simulink model "Masse_MultirotorSimHinf"  (R2018b)
settings: Solver=VariableStepAuto  StartTime=0.0  StopTime=Simulation.T_END  MaxStep=Simulation.TS_MAX  RelTol=1e-3  EnableMultiTasking=on
PreLoadFcn:
  | % InitializeParameters;
undefined symbols (not defined in the file): Aero, armed, ctrl_state, INIT_PARAM_VECTOR, Initial, K_i, K_p, Motor, mpc_att_sp, mpc_ctrl_state, mpc_manual, mpc_pos_sp_triplet, mpc_vehicle_land_detected, mpc_vehicle_status, Simulation, SOF1, SOF2, Uav, Upsilon, v_att_sp, v_control_mode
libraries: simulink_extras x9, simulink x6, dspstat3 x1, Px4Library x1
(part 4 of 11)

== matlab function Masse_MultirotorSimHinf/Sensor Model/local_position_estimator/local_position_estimator ==
  data: time input; selfVecIn input; selfVecOut output; LPE_SAMPLING_PERIOD parameter
function selfVecOut  = lpeMain( time, selfVecIn, LPE_SAMPLING_PERIOD )
%#codegen
	self = DecodeSelf( selfVecIn );
	self = LocalPositionEstimator( self, time*1e6, LPE_SAMPLING_PERIOD );
	selfVecOut = EncodeSelf( self );
end

function self = DecodeSelf( selfVecIn )
	% Variable assignment
	                                  self.A        = zeros(10,10);
	                                  self.A( 1, 1) = selfVecIn(  1);
	                                  self.A( 1, 2) = selfVecIn(  2);
	                                  self.A( 1, 3) = selfVecIn(  3);
	                                  self.A( 1, 4) = selfVecIn(  4);
	                                  self.A( 1, 5) = selfVecIn(  5);
	                                  self.A( 1, 6) = selfVecIn(  6);
	                                  self.A( 1, 7) = selfVecIn(  7);
	                                  self.A( 1, 8) = selfVecIn(  8);
	                                  self.A( 1, 9) = selfVecIn(  9);
	                                  self.A( 1,10) = selfVecIn( 10);
	                                  self.A( 2, 1) = selfVecIn( 11);
	                                  self.A( 2, 2) = selfVecIn( 12);
	                                  self.A( 2, 3) = selfVecIn( 13);
	                                  self.A( 2, 4) = selfVecIn( 14);
	                                  self.A( 2, 5) = selfVecIn( 15);
	                                  self.A( 2, 6) = selfVecIn( 16);
	                                  self.A( 2, 7) = selfVecIn( 17);
	                                  self.A( 2, 8) = selfVecIn( 18);
	                                  self.A( 2, 9) = selfVecIn( 19);
	                                  self.A( 2,10) = selfVecIn( 20);
	                                  self.A( 3, 1) = selfVecIn( 21);
	                                  self.A( 3, 2) = selfVecIn( 22);
	                                  self.A( 3, 3) = selfVecIn( 23);
	                                  self.A( 3, 4) = selfVecIn( 24);
	                                  self.A( 3, 5) = selfVecIn( 25);
	                                  self.A( 3, 6) = selfVecIn( 26);
	                                  self.A( 3, 7) = selfVecIn( 27);
	                                  self.A( 3, 8) = selfVecIn( 28);
	                                  self.A( 3, 9) = selfVecIn( 29);
	                                  self.A( 3,10) = selfVecIn( 30);
	                                  self.A( 4, 1) = selfVecIn( 31);
	                                  self.A( 4, 2) = selfVecIn( 32);
	                                  self.A( 4, 3) = selfVecIn( 33);
	                                  self.A( 4, 4) = selfVecIn( 34);
	                                  self.A( 4, 5) = selfVecIn( 35);
	                                  self.A( 4, 6) = selfVecIn( 36);
	                                  self.A( 4, 7) = selfVecIn( 37);
	                                  self.A( 4, 8) = selfVecIn( 38);
	                                  self.A( 4, 9) = selfVecIn( 39);
	                                  self.A( 4,10) = selfVecIn( 40);
	                                  self.A( 5, 1) = selfVecIn( 41);
	                                  self.A( 5, 2) = selfVecIn( 42);
	                                  self.A( 5, 3) = selfVecIn( 43);
	                                  self.A( 5, 4) = selfVecIn( 44);
	                                  self.A( 5, 5) = selfVecIn( 45);
	                                  self.A( 5, 6) = selfVecIn( 46);
	                                  self.A( 5, 7) = selfVecIn( 47);
	                                  self.A( 5, 8) = selfVecIn( 48);
	                                  self.A( 5, 9) = selfVecIn( 49);
	                                  self.A( 5,10) = selfVecIn( 50);
	                                  self.A( 6, 1) = selfVecIn( 51);
	                                  self.A( 6, 2) = selfVecIn( 52);
	                                  self.A( 6, 3) = selfVecIn( 53);
	                                  self.A( 6, 4) = selfVecIn( 54);
	                                  self.A( 6, 5) = selfVecIn( 55);
	                                  self.A( 6, 6) = selfVecIn( 56);
	                                  self.A( 6, 7) = selfVecIn( 57);
	                                  self.A( 6, 8) = selfVecIn( 58);
	                                  self.A( 6, 9) = selfVecIn( 59);
	                                  self.A( 6,10) = selfVecIn( 60);
	                                  self.A( 7, 1) = selfVecIn( 61);
	                                  self.A( 7, 2) = selfVecIn( 62);
	                                  self.A( 7, 3) = selfVecIn( 63);
	                                  self.A( 7, 4) = selfVecIn( 64);
	                                  self.A( 7, 5) = selfVecIn( 65);
	                                  self.A( 7, 6) = selfVecIn( 66);
	                                  self.A( 7, 7) = selfVecIn( 67);
	                                  self.A( 7, 8) = selfVecIn( 68);
	                                  self.A( 7, 9) = selfVecIn( 69);
	                                  self.A( 7,10) = selfVecIn( 70);
	                                  self.A( 8, 1) = selfVecIn( 71);
	                                  self.A( 8, 2) = selfVecIn( 72);
	                                  self.A( 8, 3) = selfVecIn( 73);
	                                  self.A( 8, 4) = selfVecIn( 74);
	                                  self.A( 8, 5) = selfVecIn( 75);
	                                  self.A( 8, 6) = selfVecIn( 76);
	                                  self.A( 8, 7) = selfVecIn( 77);
	                                  self.A( 8, 8) = selfVecIn( 78);
	                                  self.A( 8, 9) = selfVecIn( 79);
	                                  self.A( 8,10) = selfVecIn( 80);
	                                  self.A( 9, 1) = selfVecIn( 81);
	                                  self.A( 9, 2) = selfVecIn( 82);
	                                  self.A( 9, 3) = selfVecIn( 83);
	                                  self.A( 9, 4) = selfVecIn( 84);
	                                  self.A( 9, 5) = selfVecIn( 85);
	                                  self.A( 9, 6) = selfVecIn( 86);
	                                  self.A( 9, 7) = selfVecIn( 87);
	                                  self.A( 9, 8) = selfVecIn( 88);
	                                  self.A( 9, 9) = selfVecIn( 89);
	                                  self.A( 9,10) = selfVecIn( 90);
	                                  self.A(10, 1) = selfVecIn( 91);
	                                  self.A(10, 2) = selfVecIn( 92);
	                                  self.A(10, 3) = selfVecIn( 93);
	                                  self.A(10, 4) = selfVecIn( 94);
	                                  self.A(10, 5) = selfVecIn( 95);
	                                  self.A(10, 6) = selfVecIn( 96);
	                                  self.A(10, 7) = selfVecIn( 97);
	                                  self.A(10, 8) = selfVecIn( 98);
	                                  self.A(10, 9) = selfVecIn( 99);
	                                  self.A(10,10) = selfVecIn(100);
	                                  self.B        = zeros(10, 3);
	                                  self.B( 1, 1) = selfVecIn(101);
	                                  self.B( 1, 2) = selfVecIn(102);
	                                  self.B( 1, 3) = selfVecIn(103);
	                                  self.B( 2, 1) = selfVecIn(104);
	                                  self.B( 2, 2) = selfVecIn(105);
	                                  self.B( 2, 3) = selfVecIn(106);
	                                  self.B( 3, 1) = selfVecIn(107);
	                                  self.B( 3, 2) = selfVecIn(108);
	                                  self.B( 3, 3) = selfVecIn(109);
	                                  self.B( 4, 1) = selfVecIn(110);
	                                  self.B( 4, 2) = selfVecIn(111);
	                                  self.B( 4, 3) = selfVecIn(112);
	                                  self.B( 5, 1) = selfVecIn(113);
	                                  self.B( 5, 2) = selfVecIn(114);
	                                  self.B( 5, 3) = selfVecIn(115);
	                                  self.B( 6, 1) = selfVecIn(116);
	                                  self.B( 6, 2) = selfVecIn(117);
	                                  self.B( 6, 3) = selfVecIn(118);
	                                  self.B( 7, 1) = selfVecIn(119);
	                                  self.B( 7, 2) = selfVecIn(120);
	                                  self.B( 7, 3) = selfVecIn(121);
	                                  self.B( 8, 1) = selfVecIn(122);
	                                  self.B( 8, 2) = selfVecIn(123);
	                                  self.B( 8, 3) = selfVecIn(124);
	                                  self.B( 9, 1) = selfVecIn(125);
	                                  self.B( 9, 2) = selfVecIn(126);
	                                  self.B( 9, 3) = selfVecIn(127);
	                                  self.B(10, 1) = selfVecIn(128);
	                                  self.B(10, 2) = selfVecIn(129);
	                                  self.B(10, 3) = selfVecIn(130);
	                         self.BETA_TABLE        = zeros( 7, 1);
	                         self.BETA_TABLE( 1, 1) = selfVecIn(131);
	                         self.BETA_TABLE( 2, 1) = selfVecIn(132);
	                         self.BETA_TABLE( 3, 1) = selfVecIn(133);
	                         self.BETA_TABLE( 4, 1) = selfVecIn(134);
	                         self.BETA_TABLE( 5, 1) = selfVecIn(135);
	                         self.BETA_TABLE( 6, 1) = selfVecIn(136);
	                         self.BETA_TABLE( 7, 1) = selfVecIn(137);
	                           self.BIAS_MAX        = selfVecIn(138);
	                self.EST_STDDEV_TZ_VALID        = selfVecIn(139);
	                self.EST_STDDEV_XY_VALID        = selfVecIn(140);
	                 self.EST_STDDEV_Z_VALID        = selfVecIn(141);
	                             self.EST_TZ        = uint8(selfVecIn(142));
	                             self.EST_XY        = uint8(selfVecIn(143));
	                              self.EST_Z        = uint8(selfVecIn(144));
	                          self.FUSE_BARO        = uint8(selfVecIn(145));
	                          self.FUSE_FLOW        = uint8(selfVecIn(146));
	                self.FUSE_FLOW_GYRO_COMP        = uint8(selfVecIn(147));
	                           self.FUSE_GPS        = uint8(selfVecIn(148));
	                          self.FUSE_LAND        = uint8(selfVecIn(149));
	                     self.FUSE_PUB_AGL_Z        = uint8(selfVecIn(150));
	                       self.FUSE_VIS_POS        = uint8(selfVecIn(151));
	                       self.FUSE_VIS_YAW        = uint8(selfVecIn(152));
	                          self.HIST_STEP        = selfVecIn(153);
	                          self.LAND_RATE        = selfVecIn(154);
	                                  self.P        = zeros(10,10);
	                                  self.P( 1, 1) = selfVecIn(155);
	                                  self.P( 1, 2) = selfVecIn(156);
	                                  self.P( 1, 3) = selfVecIn(157);
	                                  self.P( 1, 4) = selfVecIn(158);
	                                  self.P( 1, 5) = selfVecIn(159);
	                                  self.P( 1, 6) = selfVecIn(160);
	                                  self.P( 1, 7) = selfVecIn(161);
	                                  self.P( 1, 8) = selfVecIn(162);
	                                  self.P( 1, 9) = selfVecIn(163);
	                                  self.P( 1,10) = selfVecIn(164);
	                                  self.P( 2, 1) = selfVecIn(165);
	                                  self.P( 2, 2) = selfVecIn(166);
	                                  self.P( 2, 3) = selfVecIn(167);
	                                  self.P( 2, 4) = selfVecIn(168);
	                                  self.P( 2, 5) = selfVecIn(169);
	                                  self.P( 2, 6) = selfVecIn(170);
	                                  self.P( 2, 7) = selfVecIn(171);
	                                  self.P( 2, 8) = selfVecIn(172);
	                                  self.P( 2, 9) = selfVecIn(173);
	                                  self.P( 2,10) = selfVecIn(174);
	                                  self.P( 3, 1) = selfVecIn(175);
	                                  self.P( 3, 2) = selfVecIn(176);
	                                  self.P( 3, 3) = selfVecIn(177);
	                                  self.P( 3, 4) = selfVecIn(178);
	                                  self.P( 3, 5) = selfVecIn(179);
	                                  self.P( 3, 6) = selfVecIn(180);
	                                  self.P( 3, 7) = selfVecIn(181);
	                                  self.P( 3, 8) = selfVecIn(182);
	                                  self.P( 3, 9) = selfVecIn(183);
	                                  self.P( 3,10) = selfVecIn(184);
	                                  self.P( 4, 1) = selfVecIn(185);
	                                  self.P( 4, 2) = selfVecIn(186);
	                                  self.P( 4, 3) = selfVecIn(187);
	                                  self.P( 4, 4) = selfVecIn(188);
	                                  self.P( 4, 5) = selfVecIn(189);
	                                  self.P( 4, 6) = selfVecIn(190);
	                                  self.P( 4, 7) = selfVecIn(191);
	                                  self.P( 4, 8) = selfVecIn(192);
	                                  self.P( 4, 9) = selfVecIn(193);
	                                  self.P( 4,10) = selfVecIn(194);
	                                  self.P( 5, 1) = selfVecIn(195);
	                                  self.P( 5, 2) = selfVecIn(196);
	                                  self.P( 5, 3) = selfVecIn(197);
	                                  self.P( 5, 4) = selfVecIn(198);
	                                  self.P( 5, 5) = selfVecIn(199);
	                                  self.P( 5, 6) = selfVecIn(200);
	                                  self.P( 5, 7) = selfVecIn(201);
	                                  self.P( 5, 8) = selfVecIn(202);
	                                  self.P( 5, 9) = selfVecIn(203);
	                                  self.P( 5,10) = selfVecIn(204);
	                                  self.P( 6, 1) = selfVecIn(205);
	                                  self.P( 6, 2) = selfVecIn(206);
	                                  self.P( 6, 3) = selfVecIn(207);
	                                  self.P( 6, 4) = selfVecIn(208);
	                                  self.P( 6, 5) = selfVecIn(209);
	                                  self.P( 6, 6) = selfVecIn(210);
	                                  self.P( 6, 7) = selfVecIn(211);
	                                  self.P( 6, 8) = selfVecIn(212);
	                                  self.P( 6, 9) = selfVecIn(213);
	                                  self.P( 6,10) = selfVecIn(214);
	                                  self.P( 7, 1) = selfVecIn(215);
	                                  self.P( 7, 2) = selfVecIn(216);
	                                  self.P( 7, 3) = selfVecIn(217);
	                                  self.P( 7, 4) = selfVecIn(218);
	                                  self.P( 7, 5) = selfVecIn(219);
	                                  self.P( 7, 6) = selfVecIn(220);
	                                  self.P( 7, 7) = selfVecIn(221);
	                                  self.P( 7, 8) = selfVecIn(222);
	                                  self.P( 7, 9) = selfVecIn(223);
	                                  self.P( 7,10) = selfVecIn(224);
	                                  self.P( 8, 1) = selfVecIn(225);
	                                  self.P( 8, 2) = selfVecIn(226);
	                                  self.P( 8, 3) = selfVecIn(227);
	                                  self.P( 8, 4) = selfVecIn(228);
	                                  self.P( 8, 5) = selfVecIn(229);
	                                  self.P( 8, 6) = selfVecIn(230);
	                                  self.P( 8, 7) = selfVecIn(231);
	                                  self.P( 8, 8) = selfVecIn(232);
	                                  self.P( 8, 9) = selfVecIn(233);
	                                  self.P( 8,10) = selfVecIn(234);
	                                  self.P( 9, 1) = selfVecIn(235);
	                                  self.P( 9, 2) = selfVecIn(236);
	                                  self.P( 9, 3) = selfVecIn(237);
	                                  self.P( 9, 4) = selfVecIn(238);
	                                  self.P( 9, 5) = selfVecIn(239);
	                                  self.P( 9, 6) = selfVecIn(240);
	                                  self.P( 9, 7) = selfVecIn(241);
	                                  self.P( 9, 8) = selfVecIn(242);
	                                  self.P( 9, 9) = selfVecIn(243);
	                                  self.P( 9,10) = selfVecIn(244);
	                                  self.P(10, 1) = selfVecIn(245);
	                                  self.P(10, 2) = selfVecIn(246);
	                                  self.P(10, 3) = selfVecIn(247);
	                                  self.P(10, 4) = selfVecIn(248);
	                                  self.P(10, 5) = selfVecIn(249);
	                                  self.P(10, 6) = selfVecIn(250);
	                                  self.P(10, 7) = selfVecIn(251);
	                                  self.P(10, 8) = selfVecIn(252);
	                                  self.P(10, 9) = selfVecIn(253);
	                                  self.P(10,10) = selfVecIn(254);
	                              self.P_MAX        = selfVecIn(255);
	                                  self.Q        = zeros(10,10);
	                                  self.Q( 1, 1) = selfVecIn(256);
	                                  self.Q( 1, 2) = selfVecIn(257);
	                                  self.Q( 1, 3) = selfVecIn(258);
	                                  self.Q( 1, 4) = selfVecIn(259);
	                                  self.Q( 1, 5) = selfVecIn(260);
	                                  self.Q( 1, 6) = selfVecIn(261);
	                                  self.Q( 1, 7) = selfVecIn(262);
	                                  self.Q( 1, 8) = selfVecIn(263);
	                                  self.Q( 1, 9) = selfVecIn(264);
	                                  self.Q( 1,10) = selfVecIn(265);
	                                  self.Q( 2, 1) = selfVecIn(266);
	                                  self.Q( 2, 2) = selfVecIn(267);
	                                  self.Q( 2, 3) = selfVecIn(268);
	                                  self.Q( 2, 4) = selfVecIn(269);
	                                  self.Q( 2, 5) = selfVecIn(270);
	                                  self.Q( 2, 6) = selfVecIn(271);
	                                  self.Q( 2, 7) = selfVecIn(272);
	                                  self.Q( 2, 8) = selfVecIn(273);
	                                  self.Q( 2, 9) = selfVecIn(274);
	                                  self.Q( 2,10) = selfVecIn(275);
	                                  self.Q( 3, 1) = selfVecIn(276);
	                                  self.Q( 3, 2) = selfVecIn(277);
	                                  self.Q( 3, 3) = selfVecIn(278);
	                                  self.Q( 3, 4) = selfVecIn(279);
	                                  self.Q( 3, 5) = selfVecIn(280);
	                                  self.Q( 3, 6) = selfVecIn(281);
	                                  self.Q( 3, 7) = selfVecIn(282);
	                                  self.Q( 3, 8) = selfVecIn(283);
	                                  self.Q( 3, 9) = selfVecIn(284);
	                                  self.Q( 3,10) = selfVecIn(285);
	                                  self.Q( 4, 1) = selfVecIn(286);
	                                  self.Q( 4, 2) = selfVecIn(287);
	                                  self.Q( 4, 3) = selfVecIn(288);
	                                  self.Q( 4, 4) = selfVecIn(289);
	                                  self.Q( 4, 5) = selfVecIn(290);
	                                  self.Q( 4, 6) = selfVecIn(291);
	                                  self.Q( 4, 7) = selfVecIn(292);
	                                  self.Q( 4, 8) = selfVecIn(293);
	                                  self.Q( 4, 9) = selfVecIn(294);
	                                  self.Q( 4,10) = selfVecIn(295);
	                                  self.Q( 5, 1) = selfVecIn(296);
	                                  self.Q( 5, 2) = selfVecIn(297);
	                                  self.Q( 5, 3) = selfVecIn(298);
	                                  self.Q( 5, 4) = selfVecIn(299);
	                                  self.Q( 5, 5) = selfVecIn(300);
	                                  self.Q( 5, 6) = selfVecIn(301);
	                                  self.Q( 5, 7) = selfVecIn(302);
	                                  self.Q( 5, 8) = selfVecIn(303);
	                                  self.Q( 5, 9) = selfVecIn(304);
	                                  self.Q( 5,10) = selfVecIn(305);
	                                  self.Q( 6, 1) = selfVecIn(306);
	                                  self.Q( 6, 2) = selfVecIn(307);
	                                  self.Q( 6, 3) = selfVecIn(308);
	                                  self.Q( 6, 4) = selfVecIn(309);
	                                  self.Q( 6, 5) = selfVecIn(310);
	                                  self.Q( 6, 6) = selfVecIn(311);
	                                  self.Q( 6, 7) = selfVecIn(312);
	                                  self.Q( 6, 8) = selfVecIn(313);
	                                  self.Q( 6, 9) = selfVecIn(314);
	                                  self.Q( 6,10) = selfVecIn(315);
	                                  self.Q( 7, 1) = selfVecIn(316);
	                                  self.Q( 7, 2) = selfVecIn(317);
	                                  self.Q( 7, 3) = selfVecIn(318);
	                                  self.Q( 7, 4) = selfVecIn(319);
	                                  self.Q( 7, 5) = selfVecIn(320);
	                                  self.Q( 7, 6) = selfVecIn(321);
	                                  self.Q( 7, 7) = selfVecIn(322);
	                                  self.Q( 7, 8) = selfVecIn(323);
	                                  self.Q( 7, 9) = selfVecIn(324);
	                                  self.Q( 7,10) = selfVecIn(325);
	                                  self.Q( 8, 1) = selfVecIn(326);
	                                  self.Q( 8, 2) = selfVecIn(327);
	                                  self.Q( 8, 3) = selfVecIn(328);
	                                  self.Q( 8, 4) = selfVecIn(329);
	                                  self.Q( 8, 5) = selfVecIn(330);
	                                  self.Q( 8, 6) = selfVecIn(331);
	                                  self.Q( 8, 7) = selfVecIn(332);
	                                  self.Q( 8, 8) = selfVecIn(333);
	                                  self.Q( 8, 9) = selfVecIn(334);
	                                  self.Q( 8,10) = selfVecIn(335);
	                                  self.Q( 9, 1) = selfVecIn(336);
	                                  self.Q( 9, 2) = selfVecIn(337);
	                                  self.Q( 9, 3) = selfVecIn(338);
	                                  self.Q( 9, 4) = selfVecIn(339);
	                                  self.Q( 9, 5) = selfVecIn(340);
	                                  self.Q( 9, 6) = selfVecIn(341);
	                                  self.Q( 9, 7) = selfVecIn(342);
	                                  self.Q( 9, 8) = selfVecIn(343);
	                                  self.Q( 9, 9) = selfVecIn(344);
	                                  self.Q( 9,10) = selfVecIn(345);
	                                  self.Q(10, 1) = selfVecIn(346);
	                                  self.Q(10, 2) = selfVecIn(347);
	                                  self.Q(10, 3) = selfVecIn(348);
	                                  self.Q(10, 4) = selfVecIn(349);
	                                  self.Q(10, 5) = selfVecIn(350);
	                                  self.Q(10, 6) = selfVecIn(351);
	                                  self.Q(10, 7) = selfVecIn(352);
	                                  self.Q(10, 8) = selfVecIn(353);
	                                  self.Q(10, 9) = selfVecIn(354);
	                                  self.Q(10,10) = selfVecIn(355);
	                                  self.R        = zeros( 3, 3);
	                                  self.R( 1, 1) = selfVecIn(356);
	                                  self.R( 1, 2) = selfVecIn(357);
	                                  self.R( 1, 3) = selfVecIn(358);
	                                  self.R( 2, 1) = selfVecIn(359);
	                                  self.R( 2, 2) = selfVecIn(360);
	                                  self.R( 2, 3) = selfVecIn(361);
	                                  self.R( 3, 1) = selfVecIn(362);
	                                  self.R( 3, 2) = selfVecIn(363);
	                                  self.R( 3, 3) = selfVecIn(364);
	                              self.R_att        = zeros( 3, 3);
	                              self.R_att( 1, 1) = selfVecIn(365);
	                              self.R_att( 1, 2) = selfVecIn(366);
	                              self.R_att( 1, 3) = selfVecIn(367);
	                              self.R_att( 2, 1) = selfVecIn(368);
	                              self.R_att( 2, 2) = selfVecIn(369);
	                              self.R_att( 2, 3) = selfVecIn(370);
	                              self.R_att( 3, 1) = selfVecIn(371);
	                              self.R_att( 3, 2) = selfVecIn(372);
	                              self.R_att( 3, 3) = selfVecIn(373);
	                        self.SENSOR_BARO        = uint8(selfVecIn(374));
	                        self.SENSOR_FLOW        = uint8(selfVecIn(375));
	                         self.SENSOR_GPS        = uint8(selfVecIn(376));
	                        self.SENSOR_LAND        = uint8(selfVecIn(377));
	                       self.SENSOR_LIDAR        = uint8(selfVecIn(378));
	                       self.SENSOR_MOCAP        = uint8(selfVecIn(379));
	                       self.SENSOR_SONAR        = uint8(selfVecIn(380));
	                      self.SENSOR_VISION        = uint8(selfVecIn(381));
	                    self.accel_xy_stddev        = selfVecIn(382);
	                    self.accel_xy_stddev        = selfVecIn(383);
	                     self.accel_z_stddev        = selfVecIn(384);
	                     self.accel_z_stddev        = selfVecIn(385);
	                      self.aglLowPass.dt        = selfVecIn(386);
	                    self.aglLowPass.fcut        = selfVecIn(387);
	                   self.aglLowPass.state        = selfVecIn(388);
	                          self.altOrigin        = selfVecIn(389);
	               self.altOriginInitialized        = selfVecIn(390);
	                      self.baroAltOrigin        = selfVecIn(391);
	                    self.baroStats.count        = selfVecIn(392);
	                    self.baroStats.total        = selfVecIn(393);
	                        self.baro_stddev        = selfVecIn(394);
	                                 self.dt        = selfVecIn(395);
	               self.estimatorInitialized        = uint8(selfVecIn(396));
	                                self.eul        = zeros( 3, 1);
	                                self.eul( 1, 1) = selfVecIn(397);
	                                self.eul( 2, 1) = selfVecIn(398);
	                                self.eul( 3, 1) = selfVecIn(399);
	                        self.fake_origin        = selfVecIn(400);
	                         self.flowQStats        = selfVecIn(401);
	              self.flow_gyro_x_high_pass        = selfVecIn(402);
	              self.flow_gyro_y_high_pass        = selfVecIn(403);
	                         self.flow_min_q        = selfVecIn(404);
	                             self.flow_r        = selfVecIn(405);
	                            self.flow_rr        = selfVecIn(406);
	                         self.flow_scale        = selfVecIn(407);
	                      self.flow_z_offset        = selfVecIn(408);
	                             self.fusion        = uint8(selfVecIn(409));
	                           self.gpsStats        = selfVecIn(410);
	                          self.gps_delay        = selfVecIn(411);
	                        self.gps_eph_max        = selfVecIn(412);
	                        self.gps_epv_max        = selfVecIn(413);
	                     self.gps_vxy_stddev        = selfVecIn(414);
	                      self.gps_vz_stddev        = selfVecIn(415);
	                      self.gps_xy_stddev        = selfVecIn(416);
	                       self.gps_z_stddev        = selfVecIn(417);
	                    self.init_origin_lat        = selfVecIn(418);
	                    self.init_origin_lon        = selfVecIn(419);
	                        self.initialized        = selfVecIn(420);
	                          self.landCount        = selfVecIn(421);
	                    self.land_vxy_stddev        = selfVecIn(422);
	                      self.land_z_stddev        = selfVecIn(423);
	                     self.lastArmedState        = selfVecIn(424);
	                     self.lidar_z_offset        = selfVecIn(425);
	                     self.lidar_z_stddev        = selfVecIn(426);
	                  self.map_ref.init_done        = selfVecIn(427);
	                    self.map_ref.lat_rad        = selfVecIn(428);
	                    self.map_ref.lon_rad        = selfVecIn(429);
	                    self.map_ref.sin_lat        = selfVecIn(430);
	                    self.map_ref.cos_lat        = selfVecIn(431);
	                  self.map_ref.timestamp        = selfVecIn(432);
	                   self.mocapStats.count        = selfVecIn(433);
	                     self.mocap_p_stddev        = selfVecIn(434);
	                 self.pn_b_noise_density        = selfVecIn(435);
	                 self.pn_p_noise_density        = selfVecIn(436);
	                 self.pn_t_noise_density        = selfVecIn(437);
	                 self.pn_v_noise_density        = selfVecIn(438);
	         self.pub_est_status.covariances        = zeros(10, 1);
	         self.pub_est_status.covariances( 1, 1) = selfVecIn(439);
	         self.pub_est_status.covariances( 2, 1) = selfVecIn(440);
	         self.pub_est_status.covariances( 3, 1) = selfVecIn(441);
	         self.pub_est_status.covariances( 4, 1) = selfVecIn(442);
	         self.pub_est_status.covariances( 5, 1) = selfVecIn(443);
	         self.pub_est_status.covariances( 6, 1) = selfVecIn(444);
	         self.pub_est_status.covariances( 7, 1) = selfVecIn(445);
	         self.pub_est_status.covariances( 8, 1) = selfVecIn(446);
	         self.pub_est_status.covariances( 9, 1) = selfVecIn(447);
	         self.pub_est_status.covariances(10, 1) = selfVecIn(448);
	        self.pub_est_status.health_flags        = uint8(selfVecIn(449));
	            self.pub_est_status.n_states        = selfVecIn(450);
	           self.pub_est_status.nan_flags        = uint8(selfVecIn(451));
	  self.pub_est_status.pos_horiz_accuracy        = selfVecIn(452);
	   self.pub_est_status.pos_vert_accuracy        = selfVecIn(453);
	              self.pub_est_status.states        = zeros(10, 1);
	              self.pub_est_status.states( 1, 1) = selfVecIn(454);
	              self.pub_est_status.states( 2, 1) = selfVecIn(455);
	              self.pub_est_status.states( 3, 1) = selfVecIn(456);
	              self.pub_est_status.states( 4, 1) = selfVecIn(457);
	              self.pub_est_status.states( 5, 1) = selfVecIn(458);
	              self.pub_est_status.states( 6, 1) = selfVecIn(459);
	              self.pub_est_status.states( 7, 1) = selfVecIn(460);
	              self.pub_est_status.states( 8, 1) = selfVecIn(461);
	              self.pub_est_status.states( 9, 1) = selfVecIn(462);
	              self.pub_est_status.states(10, 1) = selfVecIn(463);
	       self.pub_est_status.timeout_flags        = uint8(selfVecIn(464));
	           self.pub_est_status.timestamp        = selfVecIn(465);
	                       self.pub_gpos.alt        = selfVecIn(466);
	            self.pub_gpos.dead_reckoning        = selfVecIn(467);
	                       self.pub_gpos.eph        = selfVecIn(468);
	                       self.pub_gpos.epv        = selfVecIn(469);
	                       self.pub_gpos.evh        = selfVecIn(470);
	                       self.pub_gpos.evv        = selfVecIn(471);
	                       self.pub_gpos.lat        = selfVecIn(472);
	                       self.pub_gpos.lon        = selfVecIn(473);
	               self.pub_gpos.pos_d_deriv        = selfVecIn(474);
	              self.pub_gpos.pressure_alt        = selfVecIn(475);
	               self.pub_gpos.terrain_alt        = selfVecIn(476);
	         self.pub_gpos.terrain_alt_valid        = selfVecIn(477);
	             self.pub_gpos.time_utc_usec        = selfVecIn(478);
	                 self.pub_gpos.timestamp        = selfVecIn(479);
	                     self.pub_gpos.vel_n        = selfVecIn(480);
	                     self.pub_gpos.vel_e        = selfVecIn(481);
	                     self.pub_gpos.vel_d        = selfVecIn(482);
	                       self.pub_gpos.yaw        = selfVecIn(483);
	               self.pub_innov.hagl_innov        = selfVecIn(484);
	           self.pub_innov.hagl_innov_var        = selfVecIn(485);
	               self.pub_lpos.dist_bottom        = selfVecIn(486);
	          self.pub_lpos.dist_bottom_rate        = selfVecIn(487);
	         self.pub_lpos.dist_bottom_valid        = selfVecIn(488);
	                       self.pub_lpos.eph        = selfVecIn(489);
	                       self.pub_lpos.epv        = selfVecIn(490);
	                       self.pub_lpos.evh        = selfVecIn(491);
	                       self.pub_lpos.evv        = selfVecIn(492);
	                   self.pub_lpos.ref_alt        = selfVecIn(493);
	                   self.pub_lpos.ref_lat        = selfVecIn(494);
	                   self.pub_lpos.ref_lon        = selfVecIn(495);
	             self.pub_lpos.ref_timestamp        = selfVecIn(496);
	  self.pub_lpos.surface_bottom_timestamp        = selfVecIn(497);
	                 self.pub_lpos.timestamp        = selfVecIn(498);
	                self.pub_lpos.v_xy_valid        = selfVecIn(499);
	                 self.pub_lpos.v_z_valid        = selfVecIn(500);
	                        self.pub_lpos.vx        = selfVecIn(501);
	                        self.pub_lpos.vy        = selfVecIn(502);
	                        self.pub_lpos.vz        = selfVecIn(503);
	                         self.pub_lpos.x        = selfVecIn(504);
	                 self.pub_lpos.xy_global        = selfVecIn(505);
	                  self.pub_lpos.xy_valid        = selfVecIn(506);
	                         self.pub_lpos.y        = selfVecIn(507);
	                         self.pub_lpos.z        = selfVecIn(508);
	                   self.pub_lpos.z_deriv        = selfVecIn(509);
	                  self.pub_lpos.z_global        = selfVecIn(510);
	                   self.pub_lpos.z_valid        = selfVecIn(511);
	                       self.pub_lpos.yaw        = selfVecIn(512);
	                        self.sensorFault        = uint8(selfVecIn(513));
	                      self.sensorTimeout        = uint8(selfVecIn(514));
	                         self.sonarStats        = selfVecIn(515);
	                     self.sonar_z_offset        = selfVecIn(516);
	                     self.sonar_z_stddev        = selfVecIn(517);
	                    self.sub_armed.armed        = selfVecIn(518);
	                          self.sub_att.q        = zeros( 4, 1);
	                          self.sub_att.q( 1, 1) = selfVecIn(519);
	                          self.sub_att.q( 2, 1) = selfVecIn(520);
	                          self.sub_att.q( 3, 1) = selfVecIn(521);
	                          self.sub_att.q( 4, 1) = selfVecIn(522);
	                   self.sub_flow.updated        = selfVecIn(523);
	              self.sub_gps.time_utc_usec        = selfVecIn(524);
	                    self.sub_gps.updated        = selfVecIn(525);
	                  self.sub_land.freefall        = selfVecIn(526);
	                    self.sub_land.landed        = selfVecIn(527);
	                  self.sub_lidar.present        = selfVecIn(528);
	                  self.sub_lidar.updated        = selfVecIn(529);
	                self.sub_mocap.timestamp        = selfVecIn(530);
	                  self.sub_mocap.updated        = selfVecIn(531);
	                        self.sub_mocap.x        = selfVecIn(532);
	                        self.sub_mocap.y        = selfVecIn(533);
	                        self.sub_mocap.z        = selfVecIn(534);
	           self.sub_param_update.updated        = selfVecIn(535);
	self.sub_sensor.RELATIVE_TIMESTAMP_INVALID        = selfVecIn(536);
	      self.sub_sensor.accelerometer_m_s2        = zeros( 3, 1);
	      self.sub_sensor.accelerometer_m_s2( 1, 1) = selfVecIn(537);
	      self.sub_sensor.accelerometer_m_s2( 2, 1) = selfVecIn(538);
	      self.sub_sensor.accelerometer_m_s2( 3, 1) = selfVecIn(539);
	          self.sub_sensor.baro_alt_meter        = selfVecIn(540);
	 self.sub_sensor.baro_timestamp_relative        = selfVecIn(541);
	               self.sub_sensor.timestamp        = selfVecIn(542);
	                 self.sub_sensor.updated        = selfVecIn(543);
	                  self.sub_sonar.present        = selfVecIn(544);
	                  self.sub_sonar.updated        = selfVecIn(545);
	             self.sub_vision_pos.updated        = selfVecIn(546);
	                           self.tDelay.h        = zeros( 1,10);
	                           self.tDelay.h( 1, 1) = selfVecIn(547);
	                           self.tDelay.h( 1, 2) = selfVecIn(548);
	                           self.tDelay.h( 1, 3) = selfVecIn(549);
	                           self.tDelay.h( 1, 4) = selfVecIn(550);
	                           self.tDelay.h( 1, 5) = selfVecIn(551);
	                           self.tDelay.h( 1, 6) = selfVecIn(552);
	                           self.tDelay.h( 1, 7) = selfVecIn(553);
	                           self.tDelay.h( 1, 8) = selfVecIn(554);
	                           self.tDelay.h( 1, 9) = selfVecIn(555);
	                           self.tDelay.h( 1,10) = selfVecIn(556);
	                       self.tDelay.delay        = selfVecIn(557);
	                       self.tDelay.index        = selfVecIn(558);
	                        self.t_max_grade        = selfVecIn(559);
	                          self.timeStamp        = selfVecIn(560);
	                  self.timeStampLastBaro        = selfVecIn(561);
	                     self.time_last_baro        = selfVecIn(562);
	                     self.time_last_hist        = selfVecIn(563);
	                     self.time_last_land        = selfVecIn(564);
	                    self.time_last_mocap        = selfVecIn(565);
	                        self.time_origin        = selfVecIn(566);
	                                  self.u        = zeros( 3, 1);
	                                  self.u( 1, 1) = selfVecIn(567);
	                                  self.u( 2, 1) = selfVecIn(568);
	                                  self.u( 3, 1) = selfVecIn(569);
	                        self.visionStats        = selfVecIn(570);
	                       self.vision_delay        = selfVecIn(571);
	                   self.vision_xy_stddev        = selfVecIn(572);
	                    self.vision_z_stddev        = selfVecIn(573);
	                     self.vxy_pub_thresh        = selfVecIn(574);
	                                  self.x        = zeros(10, 1);
	                                  self.x( 1, 1) = selfVecIn(575);
	                                  self.x( 2, 1) = selfVecIn(576);
	                                  self.x( 3, 1) = selfVecIn(577);
	                                  self.x( 4, 1) = selfVecIn(578);
	                                  self.x( 5, 1) = selfVecIn(579);
	                                  self.x( 6, 1) = selfVecIn(580);
	                                  self.x( 7, 1) = selfVecIn(581);
	                                  self.x( 8, 1) = selfVecIn(582);
	                                  self.x( 9, 1) = selfVecIn(583);
	                                  self.x(10, 1) = selfVecIn(584);
	                           self.xDelay.h        = zeros(10,10);
	                           self.xDelay.h( 1, 1) = selfVecIn(585);
	                           self.xDelay.h( 1, 2) = selfVecIn(586);
	                           self.xDelay.h( 1, 3) = selfVecIn(587);
	                           self.xDelay.h( 1, 4) = selfVecIn(588);
	                           self.xDelay.h( 1, 5) = selfVecIn(589);
	                           self.xDelay.h( 1, 6) = selfVecIn(590);
	                           self.xDelay.h( 1, 7) = selfVecIn(591);
	                           self.xDelay.h( 1, 8) = selfVecIn(592);
	                           self.xDelay.h( 1, 9) = selfVecIn(593);
	                           self.xDelay.h( 1,10) = selfVecIn(594);
	                           self.xDelay.h( 2, 1) = selfVecIn(595);
	                           self.xDelay.h( 2, 2) = selfVecIn(596);
	                           self.xDelay.h( 2, 3) = selfVecIn(597);
	                           self.xDelay.h( 2, 4) = selfVecIn(598);
	                           self.xDelay.h( 2, 5) = selfVecIn(599);
	                           self.xDelay.h( 2, 6) = selfVecIn(600);
	                           self.xDelay.h( 2, 7) = selfVecIn(601);
	                           self.xDelay.h( 2, 8) = selfVecIn(602);
	                           self.xDelay.h( 2, 9) = selfVecIn(603);
	                           self.xDelay.h( 2,10) = selfVecIn(604);
	                           self.xDelay.h( 3, 1) = selfVecIn(605);
	                           self.xDelay.h( 3, 2) = selfVecIn(606);
	                           self.xDelay.h( 3, 3) = selfVecIn(607);
	                           self.xDelay.h( 3, 4) = selfVecIn(608);
	                           self.xDelay.h( 3, 5) = selfVecIn(609);
	                           self.xDelay.h( 3, 6) = selfVecIn(610);
	                           self.xDelay.h( 3, 7) = selfVecIn(611);
	                           self.xDelay.h( 3, 8) = selfVecIn(612);
	                           self.xDelay.h( 3, 9) = selfVecIn(613);
	                           self.xDelay.h( 3,10) = selfVecIn(614);
	                           self.xDelay.h( 4, 1) = selfVecIn(615);
	                           self.xDelay.h( 4, 2) = selfVecIn(616);
	                           self.xDelay.h( 4, 3) = selfVecIn(617);
	                           self.xDelay.h( 4, 4) = selfVecIn(618);
	                           self.xDelay.h( 4, 5) = selfVecIn(619);
	                           self.xDelay.h( 4, 6) = selfVecIn(620);
	                           self.xDelay.h( 4, 7) = selfVecIn(621);
	                           self.xDelay.h( 4, 8) = selfVecIn(622);
	                           self.xDelay.h( 4, 9) = selfVecIn(623);
	                           self.xDelay.h( 4,10) = selfVecIn(624);
	                           self.xDelay.h( 5, 1) = selfVecIn(625);
	                           self.xDelay.h( 5, 2) = selfVecIn(626);
	                           self.xDelay.h( 5, 3) = selfVecIn(627);
	                           self.xDelay.h( 5, 4) = selfVecIn(628);
	                           self.xDelay.h( 5, 5) = selfVecIn(629);
	                           self.xDelay.h( 5, 6) = selfVecIn(630);
	                           self.xDelay.h( 5, 7) = selfVecIn(631);
	                           self.xDelay.h( 5, 8) = selfVecIn(632);
	                           self.xDelay.h( 5, 9) = selfVecIn(633);
	                           self.xDelay.h( 5,10) = selfVecIn(634);
	                           self.xDelay.h( 6, 1) = selfVecIn(635);
	                           self.xDelay.h( 6, 2) = selfVecIn(636);
	                           self.xDelay.h( 6, 3) = selfVecIn(637);
	                           self.xDelay.h( 6, 4) = selfVecIn(638);
	                           self.xDelay.h( 6, 5) = selfVecIn(639);
	                           self.xDelay.h( 6, 6) = selfVecIn(640);
	                           self.xDelay.h( 6, 7) = selfVecIn(641);
	                           self.xDelay.h( 6, 8) = selfVecIn(642);
	                           self.xDelay.h( 6, 9) = selfVecIn(643);
	                           self.xDelay.h( 6,10) = selfVecIn(644);
	                           self.xDelay.h( 7, 1) = selfVecIn(645);
	                           self.xDelay.h( 7, 2) = selfVecIn(646);
	                           self.xDelay.h( 7, 3) = selfVecIn(647);
	                           self.xDelay.h( 7, 4) = selfVecIn(648);
	                           self.xDelay.h( 7, 5) = selfVecIn(649);
	                           self.xDelay.h( 7, 6) = selfVecIn(650);
	                           self.xDelay.h( 7, 7) = selfVecIn(651);
	                           self.xDelay.h( 7, 8) = selfVecIn(652);
	                           self.xDelay.h( 7, 9) = selfVecIn(653);
	                           self.xDelay.h( 7,10) = selfVecIn(654);
	                           self.xDelay.h( 8, 1) = selfVecIn(655);
	                           self.xDelay.h( 8, 2) = selfVecIn(656);
	                           self.xDelay.h( 8, 3) = selfVecIn(657);
	                           self.xDelay.h( 8, 4) = selfVecIn(658);
	                           self.xDelay.h( 8, 5) = selfVecIn(659);
	                           self.xDelay.h( 8, 6) = selfVecIn(660);
	                           self.xDelay.h( 8, 7) = selfVecIn(661);
	                           self.xDelay.h( 8, 8) = selfVecIn(662);
	                           self.xDelay.h( 8, 9) = selfVecIn(663);
	                           self.xDelay.h( 8,10) = selfVecIn(664);
	                           self.xDelay.h( 9, 1) = selfVecIn(665);
	                           self.xDelay.h( 9, 2) = selfVecIn(666);
	                           self.xDelay.h( 9, 3) = selfVecIn(667);
	                           self.xDelay.h( 9, 4) = selfVecIn(668);
	                           self.xDelay.h( 9, 5) = selfVecIn(669);
	                           self.xDelay.h( 9, 6) = selfVecIn(670);
	                           self.xDelay.h( 9, 7) = selfVecIn(671);
	                           self.xDelay.h( 9, 8) = selfVecIn(672);
	                           self.xDelay.h( 9, 9) = selfVecIn(673);
	                           self.xDelay.h( 9,10) = selfVecIn(674);
	                           self.xDelay.h(10, 1) = selfVecIn(675);
	                           self.xDelay.h(10, 2) = selfVecIn(676);
	                           self.xDelay.h(10, 3) = selfVecIn(677);
	                           self.xDelay.h(10, 4) = selfVecIn(678);
	                           self.xDelay.h(10, 5) = selfVecIn(679);
	                           self.xDelay.h(10, 6) = selfVecIn(680);
	                           self.xDelay.h(10, 7) = selfVecIn(681);
	                           self.xDelay.h(10, 8) = selfVecIn(682);
	                           self.xDelay.h(10, 9) = selfVecIn(683);
	                           self.xDelay.h(10,10) = selfVecIn(684);
	                       self.xDelay.delay        = selfVecIn(685);
	                       self.xDelay.index        = selfVecIn(686);
	                        self.xLowPass.dt        = selfVecIn(687);
	                      self.xLowPass.fcut        = selfVecIn(688);
	                     self.xLowPass.state        = zeros(10, 1);
	                     self.xLowPass.state( 1, 1) = selfVecIn(689);
	                     self.xLowPass.state( 2, 1) = selfVecIn(690);
	                     self.xLowPass.state( 3, 1) = selfVecIn(691);
	                     self.xLowPass.state( 4, 1) = selfVecIn(692);
	                     self.xLowPass.state( 5, 1) = selfVecIn(693);
	                     self.xLowPass.state( 6, 1) = selfVecIn(694);
	                     self.xLowPass.state( 7, 1) = selfVecIn(695);
	                     self.xLowPass.state( 8, 1) = selfVecIn(696);
	                     self.xLowPass.state( 9, 1) = selfVecIn(697);
	                     self.xLowPass.state(10, 1) = selfVecIn(698);
	                       self.z_pub_thresh        = selfVecIn(699);
end

function selfVecOut = EncodeSelf( self )
	% Variable assignment
	selfVecOut = zeros(699, 1);
	selfVecOut(  1) =                                   self.A( 1, 1);
	selfVecOut(  2) =                                   self.A( 1, 2);
	selfVecOut(  3) =                                   self.A( 1, 3);
	selfVecOut(  4) =                                   self.A( 1, 4);
	selfVecOut(  5) =                                   self.A( 1, 5);
	selfVecOut(  6) =                                   self.A( 1, 6);
	selfVecOut(  7) =                                   self.A( 1, 7);
	selfVecOut(  8) =                                   self.A( 1, 8);
	selfVecOut(  9) =                                   self.A( 1, 9);
	selfVecOut( 10) =                                   self.A( 1,10);
	selfVecOut( 11) =                                   self.A( 2, 1);
	selfVecOut( 12) =                                   self.A( 2, 2);
	selfVecOut( 13) =                                   self.A( 2, 3);
	selfVecOut( 14) =                                   self.A( 2, 4);
	selfVecOut( 15) =                                   self.A( 2, 5);
	selfVecOut( 16) =                                   self.A( 2, 6);
	selfVecOut( 17) =                                   self.A( 2, 7);
	selfVecOut( 18) =                                   self.A( 2, 8);
	selfVecOut( 19) =                                   self.A( 2, 9);
	selfVecOut( 20) =                                   self.A( 2,10);
	selfVecOut( 21) =                                   self.A( 3, 1);
	selfVecOut( 22) =                                   self.A( 3, 2);
	selfVecOut( 23) =                                   self.A( 3, 3);
	selfVecOut( 24) =                                   self.A( 3, 4);
	selfVecOut( 25) =                                   self.A( 3, 5);
	selfVecOut( 26) =                                   self.A( 3, 6);
	selfVecOut( 27) =                                   self.A( 3, 7);
	selfVecOut( 28) =                                   self.A( 3, 8);
	selfVecOut( 29) =                                   self.A( 3, 9);
	selfVecOut( 30) =                                   self.A( 3,10);
	selfVecOut( 31) =                                   self.A( 4, 1);
	selfVecOut( 32) =                                   self.A( 4, 2);
	selfVecOut( 33) =                                   self.A( 4, 3);
	selfVecOut( 34) =                                   self.A( 4, 4);
	selfVecOut( 35) =                                   self.A( 4, 5);
	selfVecOut( 36) =                                   self.A( 4, 6);
	selfVecOut( 37) =                                   self.A( 4, 7);
	selfVecOut( 38) =                                   self.A( 4, 8);
	selfVecOut( 39) =                                   self.A( 4, 9);
	selfVecOut( 40) =                                   self.A( 4,10);
	selfVecOut( 41) =                                   self.A( 5, 1);
	selfVecOut( 42) =                                   self.A( 5, 2);
	selfVecOut( 43) =                                   self.A( 5, 3);
	selfVecOut( 44) =                                   self.A( 5, 4);
	selfVecOut( 45) =                                   self.A( 5, 5);
	selfVecOut( 46) =                                   self.A( 5, 6);
	selfVecOut( 47) =                                   self.A( 5, 7);
	selfVecOut( 48) =                                   self.A( 5, 8);
	selfVecOut( 49) =                                   self.A( 5, 9);
	selfVecOut( 50) =                                   self.A( 5,10);
	selfVecOut( 51) =                                   self.A( 6, 1);
	selfVecOut( 52) =                                   self.A( 6, 2);
	selfVecOut( 53) =                                   self.A( 6, 3);
	selfVecOut( 54) =                                   self.A( 6, 4);
	selfVecOut( 55) =                                   self.A( 6, 5);
	selfVecOut( 56) =                                   self.A( 6, 6);
	selfVecOut( 57) =                                   self.A( 6, 7);
	selfVecOut( 58) =                                   self.A( 6, 8);
	selfVecOut( 59) =                                   self.A( 6, 9);
	selfVecOut( 60) =                                   self.A( 6,10);
	selfVecOut( 61) =                                   self.A( 7, 1);
	selfVecOut( 62) =                                   self.A( 7, 2);
	selfVecOut( 63) =                                   self.A( 7, 3);
	selfVecOut( 64) =                                   self.A( 7, 4);
	selfVecOut( 65) =                                   self.A( 7, 5);
	selfVecOut( 66) =                                   self.A( 7, 6);
	selfVecOut( 67) =                                   self.A( 7, 7);
	selfVecOut( 68) =                                   self.A( 7, 8);
	selfVecOut( 69) =                                   self.A( 7, 9);
	selfVecOut( 70) =                                   self.A( 7,10);
	selfVecOut( 71) =                                   self.A( 8, 1);
	selfVecOut( 72) =                                   self.A( 8, 2);
	selfVecOut( 73) =                                   self.A( 8, 3);
	selfVecOut( 74) =                                   self.A( 8, 4);
	selfVecOut( 75) =                                   self.A( 8, 5);
	selfVecOut( 76) =                                   self.A( 8, 6);
	selfVecOut( 77) =                                   self.A( 8, 7);
	selfVecOut( 78) =                                   self.A( 8, 8);
	selfVecOut( 79) =                                   self.A( 8, 9);
	selfVecOut( 80) =                                   self.A( 8,10);
	selfVecOut( 81) =                                   self.A( 9, 1);
	selfVecOut( 82) =                                   self.A( 9, 2);
	selfVecOut( 83) =                                   self.A( 9, 3);
	selfVecOut( 84) =                                   self.A( 9, 4);
	selfVecOut( 85) =                                   self.A( 9, 5);
	selfVecOut( 86) =                                   self.A( 9, 6);
	selfVecOut( 87) =                                   self.A( 9, 7);
	selfVecOut( 88) =                                   self.A( 9, 8);
	selfVecOut( 89) =                                   self.A( 9, 9);
	selfVecOut( 90) =                                   self.A( 9,10);
	selfVecOut( 91) =                                   self.A(10, 1);
	selfVecOut( 92) =                                   self.A(10, 2);
	selfVecOut( 93) =                                   self.A(10, 3);
	selfVecOut( 94) =                                   self.A(10, 4);
	selfVecOut( 95) =                                   self.A(10, 5);
	selfVecOut( 96) =                                   self.A(10, 6);
	selfVecOut( 97) =                                   self.A(10, 7);
	selfVecOut( 98) =                                   self.A(10, 8);
	selfVecOut( 99) =                                   self.A(10, 9);
	selfVecOut(100) =                                   self.A(10,10);
	selfVecOut(101) =                                   self.B( 1, 1);
	selfVecOut(102) =                                   self.B( 1, 2);
	selfVecOut(103) =                                   self.B( 1, 3);
	selfVecOut(104) =                                   self.B( 2, 1);
	selfVecOut(105) =                                   self.B( 2, 2);
	selfVecOut(106) =                                   self.B( 2, 3);
	selfVecOut(107) =                                   self.B( 3, 1);
	selfVecOut(108) =                                   self.B( 3, 2);
	selfVecOut(109) =                                   self.B( 3, 3);
	selfVecOut(110) =                                   self.B( 4, 1);
	selfVecOut(111) =                                   self.B( 4, 2);
	selfVecOut(112) =                                   self.B( 4, 3);
	selfVecOut(113) =                                   self.B( 5, 1);
	selfVecOut(114) =                                   self.B( 5, 2);
	selfVecOut(115) =                                   self.B( 5, 3);
	selfVecOut(116) =                                   self.B( 6, 1);
	selfVecOut(117) =                                   self.B( 6, 2);
	selfVecOut(118) =                                   self.B( 6, 3);
	selfVecOut(119) =                                   self.B( 7, 1);
	selfVecOut(120) =                                   self.B( 7, 2);
	selfVecOut(121) =                                   self.B( 7, 3);
	selfVecOut(122) =                                   self.B( 8, 1);
	selfVecOut(123) =                                   self.B( 8, 2);
	selfVecOut(124) =                                   self.B( 8, 3);
	selfVecOut(125) =                                   self.B( 9, 1);
	selfVecOut(126) =                                   self.B( 9, 2);
	selfVecOut(127) =                                   self.B( 9, 3);
	selfVecOut(128) =                                   self.B(10, 1);
	selfVecOut(129) =                                   self.B(10, 2);
	selfVecOut(130) =                                   self.B(10, 3);
	selfVecOut(131) =                          self.BETA_TABLE( 1, 1);
	selfVecOut(132) =                          self.BETA_TABLE( 2, 1);
	selfVecOut(133) =                          self.BETA_TABLE( 3, 1);
	selfVecOut(134) =                          self.BETA_TABLE( 4, 1);
	selfVecOut(135) =                          self.BETA_TABLE( 5, 1);
	selfVecOut(136) =                          self.BETA_TABLE( 6, 1);
	selfVecOut(137) =                          self.BETA_TABLE( 7, 1);
	selfVecOut(138) =                            self.BIAS_MAX( 1, 1);
	selfVecOut(139) =                 self.EST_STDDEV_TZ_VALID( 1, 1);
	selfVecOut(140) =                 self.EST_STDDEV_XY_VALID( 1, 1);
	selfVecOut(141) =                  self.EST_STDDEV_Z_VALID( 1, 1);
	selfVecOut(142) = double(                      self.EST_TZ( 1, 1));
	selfVecOut(143) = double(                      self.EST_XY( 1, 1));
	selfVecOut(144) = double(                       self.EST_Z( 1, 1));
	selfVecOut(145) = double(                   self.FUSE_BARO( 1, 1));
	selfVecOut(146) = double(                   self.FUSE_FLOW( 1, 1));
	selfVecOut(147) = double(         self.FUSE_FLOW_GYRO_COMP( 1, 1));
	selfVecOut(148) = double(                    self.FUSE_GPS( 1, 1));
	selfVecOut(149) = double(                   self.FUSE_LAND( 1, 1));
	selfVecOut(150) = double(              self.FUSE_PUB_AGL_Z( 1, 1));
	selfVecOut(151) = double(                self.FUSE_VIS_POS( 1, 1));
	selfVecOut(152) = double(                self.FUSE_VIS_YAW( 1, 1));
	selfVecOut(153) =                           self.HIST_STEP( 1, 1);
	selfVecOut(154) =                           self.LAND_RATE( 1, 1);
	selfVecOut(155) =                                   self.P( 1, 1);
	selfVecOut(156) =                                   self.P( 1, 2);
	selfVecOut(157) =                                   self.P( 1, 3);
	selfVecOut(158) =                                   self.P( 1, 4);
	selfVecOut(159) =                                   self.P( 1, 5);
	selfVecOut(160) =                                   self.P( 1, 6);
	selfVecOut(161) =                                   self.P( 1, 7);
	selfVecOut(162) =                                   self.P( 1, 8);
	selfVecOut(163) =                                   self.P( 1, 9);
	selfVecOut(164) =                                   self.P( 1,10);
	selfVecOut(165) =                                   self.P( 2, 1);
	selfVecOut(166) =                                   self.P( 2, 2);
	selfVecOut(167) =                                   self.P( 2, 3);
	selfVecOut(168) =                                   self.P( 2, 4);
	selfVecOut(169) =                                   self.P( 2, 5);
	selfVecOut(170) =                                   self.P( 2, 6);
	selfVecOut(171) =                                   self.P( 2, 7);
	selfVecOut(172) =                                   self.P( 2, 8);
	selfVecOut(173) =                                   self.P( 2, 9);
	selfVecOut(174) =                                   self.P( 2,10);
	selfVecOut(175) =                                   self.P( 3, 1);
	selfVecOut(176) =                                   self.P( 3, 2);
	selfVecOut(177) =                                   self.P( 3, 3);
	selfVecOut(178) =                                   self.P( 3, 4);
	selfVecOut(179) =                                   self.P( 3, 5);
	selfVecOut(180) =                                   self.P( 3, 6);
	selfVecOut(181) =                                   self.P( 3, 7);
	selfVecOut(182) =                                   self.P( 3, 8);
	selfVecOut(183) =                                   self.P( 3, 9);
	selfVecOut(184) =                                   self.P( 3,10);
	selfVecOut(185) =                                   self.P( 4, 1);
	selfVecOut(186) =                                   self.P( 4, 2);
	selfVecOut(187) =                                   self.P( 4, 3);
	selfVecOut(188) =                                   self.P( 4, 4);
	selfVecOut(189) =                                   self.P( 4, 5);
	selfVecOut(190) =                                   self.P( 4, 6);
	selfVecOut(191) =                                   self.P( 4, 7);
	selfVecOut(192) =                                   self.P( 4, 8);
	selfVecOut(193) =                                   self.P( 4, 9);
	selfVecOut(194) =                                   self.P( 4,10);
	selfVecOut(195) =                                   self.P( 5, 1);
	selfVecOut(196) =                                   self.P( 5, 2);
	selfVecOut(197) =                                   self.P( 5, 3);
	selfVecOut(198) =                                   self.P( 5, 4);
	selfVecOut(199) =                                   self.P( 5, 5);
	selfVecOut(200) =                                   self.P( 5, 6);
	selfVecOut(201) =                                   self.P( 5, 7);
	selfVecOut(202) =                                   self.P( 5, 8);
	selfVecOut(203) =                                   self.P( 5, 9);
	selfVecOut(204) =                                   self.P( 5,10);
	selfVecOut(205) =                                   self.P( 6, 1);
	selfVecOut(206) =                                   self.P( 6, 2);
	selfVecOut(207) =                                   self.P( 6, 3);
	selfVecOut(208) =                                   self.P( 6, 4);
	selfVecOut(209) =                                   self.P( 6, 5);
	selfVecOut(210) =                                   self.P( 6, 6);
	selfVecOut(211) =                                   self.P( 6, 7);
	selfVecOut(212) =                                   self.P( 6, 8);
	selfVecOut(213) =                                   self.P( 6, 9);
	selfVecOut(214) =                                   self.P( 6,10);
	selfVecOut(215) =                                   self.P( 7, 1);
	selfVecOut(216) =                                   self.P( 7, 2);
	selfVecOut(217) =                                   self.P( 7, 3);
	selfVecOut(218) =                                   self.P( 7, 4);
	selfVecOut(219) =                                   self.P( 7, 5);
	selfVecOut(220) =                                   self.P( 7, 6);
	selfVecOut(221) =                                   self.P( 7, 7);
	selfVecOut(222) =                                   self.P( 7, 8);
	selfVecOut(223) =                                   self.P( 7, 9);
	selfVecOut(224) =                                   self.P( 7,10);
	selfVecOut(225) =                                   self.P( 8, 1);
	selfVecOut(226) =                                   self.P( 8, 2);
	selfVecOut(227) =                                   self.P( 8, 3);
	selfVecOut(228) =                                   self.P( 8, 4);
	selfVecOut(229) =                                   self.P( 8, 5);
	selfVecOut(230) =                                   self.P( 8, 6);
	selfVecOut(231) =                                   self.P( 8, 7);
	selfVecOut(232) =                                   self.P( 8, 8);
	selfVecOut(233) =                                   self.P( 8, 9);
	selfVecOut(234) =                                   self.P( 8,10);
	selfVecOut(235) =                                   self.P( 9, 1);
	selfVecOut(236) =                                   self.P( 9, 2);
	selfVecOut(237) =                                   self.P( 9, 3);
	selfVecOut(238) =                                   self.P( 9, 4);
	selfVecOut(239) =                                   self.P( 9, 5);
	selfVecOut(240) =                                   self.P( 9, 6);
	selfVecOut(241) =                                   self.P( 9, 7);
	selfVecOut(242) =                                   self.P( 9, 8);
	selfVecOut(243) =                                   self.P( 9, 9);
	selfVecOut(244) =                                   self.P( 9,10);
	selfVecOut(245) =                                   self.P(10, 1);
	selfVecOut(246) =                                   self.P(10, 2);
	selfVecOut(247) =                                   self.P(10, 3);
	selfVecOut(248) =                                   self.P(10, 4);
	selfVecOut(249) =                                   self.P(10, 5);
	selfVecOut(250) =                                   self.P(10, 6);
	selfVecOut(251) =                                   self.P(10, 7);
	selfVecOut(252) =                                   self.P(10, 8);
	selfVecOut(253) =                                   self.P(10, 9);
	selfVecOut(254) =                                   self.P(10,10);
	selfVecOut(255) =                               self.P_MAX( 1, 1);
	selfVecOut(256) =                                   self.Q( 1, 1);
	selfVecOut(257) =                                   self.Q( 1, 2);
	selfVecOut(258) =                                   self.Q( 1, 3);
	selfVecOut(259) =                                   self.Q( 1, 4);
	selfVecOut(260) =                                   self.Q( 1, 5);
	selfVecOut(261) =                                   self.Q( 1, 6);
	selfVecOut(262) =                                   self.Q( 1, 7);
	selfVecOut(263) =                                   self.Q( 1, 8);
	selfVecOut(264) =                                   self.Q( 1, 9);
	selfVecOut(265) =                                   self.Q( 1,10);
	selfVecOut(266) =                                   self.Q( 2, 1);
	selfVecOut(267) =                                   self.Q( 2, 2);
	selfVecOut(268) =                                   self.Q( 2, 3);
	selfVecOut(269) =                                   self.Q( 2, 4);
	selfVecOut(270) =                                   self.Q( 2, 5);
	selfVecOut(271) =                                   self.Q( 2, 6);
	selfVecOut(272) =                                   self.Q( 2, 7);
	selfVecOut(273) =                                   self.Q( 2, 8);
	selfVecOut(274) =                                   self.Q( 2, 9);
	selfVecOut(275) =                                   self.Q( 2,10);
	selfVecOut(276) =                                   self.Q( 3, 1);
	selfVecOut(277) =                                   self.Q( 3, 2);
	selfVecOut(278) =                                   self.Q( 3, 3);
	selfVecOut(279) =                                   self.Q( 3, 4);
	selfVecOut(280) =                                   self.Q( 3, 5);
	selfVecOut(281) =                                   self.Q( 3, 6);
	selfVecOut(282) =                                   self.Q( 3, 7);
	selfVecOut(283) =                                   self.Q( 3, 8);
	selfVecOut(284) =                                   self.Q( 3, 9);
	selfVecOut(285) =                                   self.Q( 3,10);
	selfVecOut(286) =                                   self.Q( 4, 1);
	selfVecOut(287) =                                   self.Q( 4, 2);
	selfVecOut(288) =                                   self.Q( 4, 3);
	selfVecOut(289) =                                   self.Q( 4, 4);
	selfVecOut(290) =                                   self.Q( 4, 5);
	selfVecOut(291) =                                   self.Q( 4, 6);
	selfVecOut(292) =                                   self.Q( 4, 7);
	selfVecOut(293) =                                   self.Q( 4, 8);
	selfVecOut(294) =                                   self.Q( 4, 9);
	selfVecOut(295) =                                   self.Q( 4,10);
	selfVecOut(296) =                                   self.Q( 5, 1);
	selfVecOut(297) =                                   self.Q( 5, 2);
	selfVecOut(298) =                                   self.Q( 5, 3);
	selfVecOut(299) =                                   self.Q( 5, 4);
	selfVecOut(300) =                                   self.Q( 5, 5);
	selfVecOut(301) =                                   self.Q( 5, 6);
	selfVecOut(302) =                                   self.Q( 5, 7);
	selfVecOut(303) =                                   self.Q( 5, 8);
	selfVecOut(304) =                                   self.Q( 5, 9);
	selfVecOut(305) =                                   self.Q( 5,10);
	selfVecOut(306) =                                   self.Q( 6, 1);
	selfVecOut(307) =                                   self.Q( 6, 2);
	selfVecOut(308) =                                   self.Q( 6, 3);
	selfVecOut(309) =                                   self.Q( 6, 4);
	selfVecOut(310) =                                   self.Q( 6, 5);
	selfVecOut(311) =                                   self.Q( 6, 6);
	selfVecOut(312) =                                   self.Q( 6, 7);
	selfVecOut(313) =                                   self.Q( 6, 8);
	selfVecOut(314) =                                   self.Q( 6, 9);
	selfVecOut(315) =                                   self.Q( 6,10);
	selfVecOut(316) =                                   self.Q( 7, 1);
	selfVecOut(317) =                                   self.Q( 7, 2);
	selfVecOut(318) =                                   self.Q( 7, 3);
	selfVecOut(319) =                                   self.Q( 7, 4);
	selfVecOut(320) =                                   self.Q( 7, 5);
	selfVecOut(321) =                                   self.Q( 7, 6);
	selfVecOut(322) =                                   self.Q( 7, 7);
	selfVecOut(323) =                                   self.Q( 7, 8);
	selfVecOut(324) =                                   self.Q( 7, 9);
	selfVecOut(325) =                                   self.Q( 7,10);
	selfVecOut(326) =                                   self.Q( 8, 1);
	selfVecOut(327) =                                   self.Q( 8, 2);
	selfVecOut(328) =                                   self.Q( 8, 3);
	selfVecOut(329) =                                   self.Q( 8, 4);
	selfVecOut(330) =                                   self.Q( 8, 5);
	selfVecOut(331) =                                   self.Q( 8, 6);
	selfVecOut(332) =                                   self.Q( 8, 7);
	selfVecOut(333) =                                   self.Q( 8, 8);
	selfVecOut(334) =                                   self.Q( 8, 9);
	selfVecOut(335) =                                   self.Q( 8,10);
	selfVecOut(336) =                                   self.Q( 9, 1);
	selfVecOut(337) =                                   self.Q( 9, 2);
	selfVecOut(338) =                                   self.Q( 9, 3);
	selfVecOut(339) =                                   self.Q( 9, 4);
	selfVecOut(340) =                                   self.Q( 9, 5);
	selfVecOut(341) =                                   self.Q( 9, 6);
	selfVecOut(342) =                                   self.Q( 9, 7);
	selfVecOut(343) =                                   self.Q( 9, 8);
	selfVecOut(344) =                                   self.Q( 9, 9);
	selfVecOut(345) =                                   self.Q( 9,10);
	selfVecOut(346) =                                   self.Q(10, 1);
	selfVecOut(347) =                                   self.Q(10, 2);
	selfVecOut(348) =                                   self.Q(10, 3);
	selfVecOut(349) =                                   self.Q(10, 4);
	selfVecOut(350) =                                   self.Q(10, 5);
	selfVecOut(351) =                                   self.Q(10, 6);
	selfVecOut(352) =                                   self.Q(10, 7);
	selfVecOut(353) =                                   self.Q(10, 8);
	selfVecOut(354) =                                   self.Q(10, 9);
	selfVecOut(355) =                                   self.Q(10,10);
	selfVecOut(356) =                                   self.R( 1, 1);
	selfVecOut(357) =                                   self.R( 1, 2);
	selfVecOut(358) =                                   self.R( 1, 3);
	selfVecOut(359) =                                   self.R( 2, 1);
	selfVecOut(360) =                                   self.R( 2, 2);
	selfVecOut(361) =                                   self.R( 2, 3);
	selfVecOut(362) =                                   self.R( 3, 1);
	selfVecOut(363) =                                   self.R( 3, 2);
	selfVecOut(364) =                                   self.R( 3, 3);
	selfVecOut(365) =                               self.R_att( 1, 1);
	selfVecOut(366) =                               self.R_att( 1, 2);
	selfVecOut(367) =                               self.R_att( 1, 3);
	selfVecOut(368) =                               self.R_att( 2, 1);
	selfVecOut(369) =                               self.R_att( 2, 2);
	selfVecOut(370) =                               self.R_att( 2, 3);
	selfVecOut(371) =                               self.R_att( 3, 1);
	selfVecOut(372) =                               self.R_att( 3, 2);
	selfVecOut(373) =                               self.R_att( 3, 3);
	selfVecOut(374) = double(                 self.SENSOR_BARO( 1, 1));
	selfVecOut(375) = double(                 self.SENSOR_FLOW( 1, 1));
	selfVecOut(376) = double(                  self.SENSOR_GPS( 1, 1));
	selfVecOut(377) = double(                 self.SENSOR_LAND( 1, 1));
	selfVecOut(378) = double(                self.SENSOR_LIDAR( 1, 1));
	selfVecOut(379) = double(                self.SENSOR_MOCAP( 1, 1));
	selfVecOut(380) = double(                self.SENSOR_SONAR( 1, 1));
	selfVecOut(381) = double(               self.SENSOR_VISION( 1, 1));
	selfVecOut(382) =                     self.accel_xy_stddev( 1, 1);
	selfVecOut(383) =                     self.accel_xy_stddev( 1, 1);
	selfVecOut(384) =                      self.accel_z_stddev( 1, 1);
	selfVecOut(385) =                      self.accel_z_stddev( 1, 1);
	selfVecOut(386) =                       self.aglLowPass.dt( 1, 1);
	selfVecOut(387) =                     self.aglLowPass.fcut( 1, 1);
	selfVecOut(388) =                    self.aglLowPass.state( 1, 1);
	selfVecOut(389) =                           self.altOrigin( 1, 1);
	selfVecOut(390) =                self.altOriginInitialized( 1, 1);
	selfVecOut(391) =                       self.baroAltOrigin( 1, 1);
	selfVecOut(392) =                     self.baroStats.count( 1, 1);
	selfVecOut(393) =                     self.baroStats.total( 1, 1);
	selfVecOut(394) =                         self.baro_stddev( 1, 1);
	selfVecOut(395) =                                  self.dt( 1, 1);
	selfVecOut(396) = double(        self.estimatorInitialized( 1, 1));
	selfVecOut(397) =                                 self.eul( 1, 1);
	selfVecOut(398) =                                 self.eul( 2, 1);
	selfVecOut(399) =                                 self.eul( 3, 1);
	selfVecOut(400) =                         self.fake_origin( 1, 1);
	selfVecOut(401) =                          self.flowQStats( 1, 1);
	selfVecOut(402) =               self.flow_gyro_x_high_pass( 1, 1);
	selfVecOut(403) =               self.flow_gyro_y_high_pass( 1, 1);
	selfVecOut(404) =                          self.flow_min_q( 1, 1);
	selfVecOut(405) =                              self.flow_r( 1, 1);
	selfVecOut(406) =                             self.flow_rr( 1, 1);
	selfVecOut(407) =                          self.flow_scale( 1, 1);
	selfVecOut(408) =                       self.flow_z_offset( 1, 1);
	selfVecOut(409) = double(                      self.fusion( 1, 1));
	selfVecOut(410) =                            self.gpsStats( 1, 1);
	selfVecOut(411) =                           self.gps_delay( 1, 1);
	selfVecOut(412) =                         self.gps_eph_max( 1, 1);
	selfVecOut(413) =                         self.gps_epv_max( 1, 1);
	selfVecOut(414) =                      self.gps_vxy_stddev( 1, 1);
	selfVecOut(415) =                       self.gps_vz_stddev( 1, 1);
	selfVecOut(416) =                       self.gps_xy_stddev( 1, 1);
	selfVecOut(417) =                        self.gps_z_stddev( 1, 1);
	selfVecOut(418) =                     self.init_origin_lat( 1, 1);
	selfVecOut(419) =                     self.init_origin_lon( 1, 1);
	selfVecOut(420) =                         self.initialized( 1, 1);
	selfVecOut(421) =                           self.landCount( 1, 1);
	selfVecOut(422) =                     self.land_vxy_stddev( 1, 1);
	selfVecOut(423) =                       self.land_z_stddev( 1, 1);
	selfVecOut(424) =                      self.lastArmedState( 1, 1);
	selfVecOut(425) =                      self.lidar_z_offset( 1, 1);
	selfVecOut(426) =                      self.lidar_z_stddev( 1, 1);
	selfVecOut(427) =                   self.map_ref.init_done( 1, 1);
	selfVecOut(428) =                     self.map_ref.lat_rad( 1, 1);
	selfVecOut(429) =                     self.map_ref.lon_rad( 1, 1);
	selfVecOut(430) =                     self.map_ref.sin_lat( 1, 1);
	selfVecOut(431) =                     self.map_ref.cos_lat( 1, 1);
	selfVecOut(432) =                   self.map_ref.timestamp( 1, 1);
	selfVecOut(433) =                    self.mocapStats.count( 1, 1);
	selfVecOut(434) =                      self.mocap_p_stddev( 1, 1);
	selfVecOut(435) =                  self.pn_b_noise_density( 1, 1);
	selfVecOut(436) =                  self.pn_p_noise_density( 1, 1);
	selfVecOut(437) =                  self.pn_t_noise_density( 1, 1);
	selfVecOut(438) =                  self.pn_v_noise_density( 1, 1);
	selfVecOut(439) =          self.pub_est_status.covariances( 1, 1);
	selfVecOut(440) =          self.pub_est_status.covariances( 2, 1);
	selfVecOut(441) =          self.pub_est_status.covariances( 3, 1);
	selfVecOut(442) =          self.pub_est_status.covariances( 4, 1);
	selfVecOut(443) =          self.pub_est_status.covariances( 5, 1);
	selfVecOut(444) =          self.pub_est_status.covariances( 6, 1);
	selfVecOut(445) =          self.pub_est_status.covariances( 7, 1);
	selfVecOut(446) =          self.pub_est_status.covariances( 8, 1);
	selfVecOut(447) =          self.pub_est_status.covariances( 9, 1);
	selfVecOut(448) =          self.pub_est_status.covariances(10, 1);
	selfVecOut(449) = double( self.pub_est_status.health_flags( 1, 1));
	selfVecOut(450) =             self.pub_est_status.n_states( 1, 1);
	selfVecOut(451) = double(    self.pub_est_status.nan_flags( 1, 1));
	selfVecOut(452) =   self.pub_est_status.pos_horiz_accuracy( 1, 1);
	selfVecOut(453) =    self.pub_est_status.pos_vert_accuracy( 1, 1);
	selfVecOut(454) =               self.pub_est_status.states( 1, 1);
	selfVecOut(455) =               self.pub_est_status.states( 2, 1);
	selfVecOut(456) =               self.pub_est_status.states( 3, 1);
	selfVecOut(457) =               self.pub_est_status.states( 4, 1);
	selfVecOut(458) =               self.pub_est_status.states( 5, 1);
	selfVecOut(459) =               self.pub_est_status.states( 6, 1);
	selfVecOut(460) =               self.pub_est_status.states( 7, 1);
	selfVecOut(461) =               self.pub_est_status.states( 8, 1);
	selfVecOut(462) =               self.pub_est_status.states( 9, 1);
	selfVecOut(463) =               self.pub_est_status.states(10, 1);
	selfVecOut(464) = double(self.pub_est_status.timeout_flags( 1, 1));
	selfVecOut(465) =            self.pub_est_status.timestamp( 1, 1);
	selfVecOut(466) =                        self.pub_gpos.alt( 1, 1);
	selfVecOut(467) =             self.pub_gpos.dead_reckoning( 1, 1);
	selfVecOut(468) =                        self.pub_gpos.eph( 1, 1);
	selfVecOut(469) =                        self.pub_gpos.epv( 1, 1);
	selfVecOut(470) =                        self.pub_gpos.evh( 1, 1);
	selfVecOut(471) =                        self.pub_gpos.evv( 1, 1);
	selfVecOut(472) =                        self.pub_gpos.lat( 1, 1);
	selfVecOut(473) =                        self.pub_gpos.lon( 1, 1);
	selfVecOut(474) =                self.pub_gpos.pos_d_deriv( 1, 1);
	selfVecOut(475) =               self.pub_gpos.pressure_alt( 1, 1);
	selfVecOut(476) =                self.pub_gpos.terrain_alt( 1, 1);
	selfVecOut(477) =          self.pub_gpos.terrain_alt_valid( 1, 1);
	selfVecOut(478) =              self.pub_gpos.time_utc_usec( 1, 1);
	selfVecOut(479) =                  self.pub_gpos.timestamp( 1, 1);
	selfVecOut(480) =                      self.pub_gpos.vel_n( 1, 1);
	selfVecOut(481) =                      self.pub_gpos.vel_e( 1, 1);
	selfVecOut(482) =                      self.pub_gpos.vel_d( 1, 1);
	selfVecOut(483) =                        self.pub_gpos.yaw( 1, 1);
	selfVecOut(484) =                self.pub_innov.hagl_innov( 1, 1);
	selfVecOut(485) =            self.pub_innov.hagl_innov_var( 1, 1);
	selfVecOut(486) =                self.pub_lpos.dist_bottom( 1, 1);
	selfVecOut(487) =           self.pub_lpos.dist_bottom_rate( 1, 1);
	selfVecOut(488) =          self.pub_lpos.dist_bottom_valid( 1, 1);
	selfVecOut(489) =                        self.pub_lpos.eph( 1, 1);
	selfVecOut(490) =                        self.pub_lpos.epv( 1, 1);
	selfVecOut(491) =                        self.pub_lpos.evh( 1, 1);
	selfVecOut(492) =                        self.pub_lpos.evv( 1, 1);
	selfVecOut(493) =                    self.pub_lpos.ref_alt( 1, 1);
	selfVecOut(494) =                    self.pub_lpos.ref_lat( 1, 1);
	selfVecOut(495) =                    self.pub_lpos.ref_lon( 1, 1);
	selfVecOut(496) =              self.pub_lpos.ref_timestamp( 1, 1);
	selfVecOut(497) =   self.pub_lpos.surface_bottom_timestamp( 1, 1);
	selfVecOut(498) =                  self.pub_lpos.timestamp( 1, 1);
	selfVecOut(499) =                 self.pub_lpos.v_xy_valid( 1, 1);
	selfVecOut(500) =                  self.pub_lpos.v_z_valid( 1, 1);
	selfVecOut(501) =                         self.pub_lpos.vx( 1, 1);
	selfVecOut(502) =                         self.pub_lpos.vy( 1, 1);
	selfVecOut(503) =                         self.pub_lpos.vz( 1, 1);
	selfVecOut(504) =                          self.pub_lpos.x( 1, 1);
	selfVecOut(505) =                  self.pub_lpos.xy_global( 1, 1);
	selfVecOut(506) =                   self.pub_lpos.xy_valid( 1, 1);
	selfVecOut(507) =                          self.pub_lpos.y( 1, 1);
	selfVecOut(508) =                          self.pub_lpos.z( 1, 1);
	selfVecOut(509) =                    self.pub_lpos.z_deriv( 1, 1);
	selfVecOut(510) =                   self.pub_lpos.z_global( 1, 1);
	selfVecOut(511) =                    self.pub_lpos.z_valid( 1, 1);
	selfVecOut(512) =                        self.pub_lpos.yaw( 1, 1);
	selfVecOut(513) = double(                 self.sensorFault( 1, 1));
	selfVecOut(514) = double(               self.sensorTimeout( 1, 1));
	selfVecOut(515) =                          self.sonarStats( 1, 1);
	selfVecOut(516) =                      self.sonar_z_offset( 1, 1);
	selfVecOut(517) =                      self.sonar_z_stddev( 1, 1);
	selfVecOut(518) =                     self.sub_armed.armed( 1, 1);
	selfVecOut(519) =                           self.sub_att.q( 1, 1);
	selfVecOut(520) =                           self.sub_att.q( 2, 1);
	selfVecOut(521) =                           self.sub_att.q( 3, 1);
	selfVecOut(522) =                           self.sub_att.q( 4, 1);
	selfVecOut(523) =                    self.sub_flow.updated( 1, 1);
	selfVecOut(524) =               self.sub_gps.time_utc_usec( 1, 1);
	selfVecOut(525) =                     self.sub_gps.updated( 1, 1);
	selfVecOut(526) =                   self.sub_land.freefall( 1, 1);
	selfVecOut(527) =                     self.sub_land.landed( 1, 1);
	selfVecOut(528) =                   self.sub_lidar.present( 1, 1);
	selfVecOut(529) =                   self.sub_lidar.updated( 1, 1);
	selfVecOut(530) =                 self.sub_mocap.timestamp( 1, 1);
	selfVecOut(531) =                   self.sub_mocap.updated( 1, 1);
	selfVecOut(532) =                         self.sub_mocap.x( 1, 1);
	selfVecOut(533) =                         self.sub_mocap.y( 1, 1);
	selfVecOut(534) =                         self.sub_mocap.z( 1, 1);
	selfVecOut(535) =            self.sub_param_update.updated( 1, 1);
	selfVecOut(536) = self.sub_sensor.RELATIVE_TIMESTAMP_INVALID( 1, 1);
	selfVecOut(537) =       self.sub_sensor.accelerometer_m_s2( 1, 1);
	selfVecOut(538) =       self.sub_sensor.accelerometer_m_s2( 2, 1);
	selfVecOut(539) =       self.sub_sensor.accelerometer_m_s2( 3, 1);
	selfVecOut(540) =           self.sub_sensor.baro_alt_meter( 1, 1);
	selfVecOut(541) =  self.sub_sensor.baro_timestamp_relative( 1, 1);
	selfVecOut(542) =                self.sub_sensor.timestamp( 1, 1);
	selfVecOut(543) =                  self.sub_sensor.updated( 1, 1);
	selfVecOut(544) =                   self.sub_sonar.present( 1, 1);
	selfVecOut(545) =                   self.sub_sonar.updated( 1, 1);
	selfVecOut(546) =              self.sub_vision_pos.updated( 1, 1);
	selfVecOut(547) =                            self.tDelay.h( 1, 1);
	selfVecOut(548) =                            self.tDelay.h( 1, 2);
	selfVecOut(549) =                            self.tDelay.h( 1, 3);
	selfVecOut(550) =                            self.tDelay.h( 1, 4);
	selfVecOut(551) =                            self.tDelay.h( 1, 5);
	selfVecOut(552) =                            self.tDelay.h( 1, 6);
	selfVecOut(553) =                            self.tDelay.h( 1, 7);
	selfVecOut(554) =                            self.tDelay.h( 1, 8);
	selfVecOut(555) =                            self.tDelay.h( 1, 9);
	selfVecOut(556) =                            self.tDelay.h( 1,10);
	selfVecOut(557) =                        self.tDelay.delay( 1, 1);
	selfVecOut(558) =                        self.tDelay.index( 1, 1);
	selfVecOut(559) =                         self.t_max_grade( 1, 1);
	selfVecOut(560) =                           self.timeStamp( 1, 1);
	selfVecOut(561) =                   self.timeStampLastBaro( 1, 1);
	selfVecOut(562) =                      self.time_last_baro( 1, 1);
	selfVecOut(563) =                      self.time_last_hist( 1, 1);
	selfVecOut(564) =                      self.time_last_land( 1, 1);
	selfVecOut(565) =                     self.time_last_mocap( 1, 1);
	selfVecOut(566) =                         self.time_origin( 1, 1);
	selfVecOut(567) =                                   self.u( 1, 1);
	selfVecOut(568) =                                   self.u( 2, 1);
	selfVecOut(569) =                                   self.u( 3, 1);
	selfVecOut(570) =                         self.visionStats( 1, 1);
	selfVecOut(571) =                        self.vision_delay( 1, 1);
	selfVecOut(572) =                    self.vision_xy_stddev( 1, 1);
	selfVecOut(573) =                     self.vision_z_stddev( 1, 1);
	selfVecOut(574) =                      self.vxy_pub_thresh( 1, 1);
	selfVecOut(575) =                                   self.x( 1, 1);
	selfVecOut(576) =                                   self.x( 2, 1);
	selfVecOut(577) =                                   self.x( 3, 1);
	selfVecOut(578) =                                   self.x( 4, 1);
	selfVecOut(579) =                                   self.x( 5, 1);
	selfVecOut(580) =                                   self.x( 6, 1);
	selfVecOut(581) =                                   self.x( 7, 1);
	selfVecOut(582) =                                   self.x( 8, 1);
	selfVecOut(583) =                                   self.x( 9, 1);
	selfVecOut(584) =                                   self.x(10, 1);
	selfVecOut(585) =                            self.xDelay.h( 1, 1);
	selfVecOut(586) =                            self.xDelay.h( 1, 2);
	selfVecOut(587) =                            self.xDelay.h( 1, 3);
	selfVecOut(588) =                            self.xDelay.h( 1, 4);
	selfVecOut(589) =                            self.xDelay.h( 1, 5);
	selfVecOut(590) =                            self.xDelay.h( 1, 6);
	selfVecOut(591) =                            self.xDelay.h( 1, 7);
	selfVecOut(592) =                            self.xDelay.h( 1, 8);
	selfVecOut(593) =                            self.xDelay.h( 1, 9);
	selfVecOut(594) =                            self.xDelay.h( 1,10);
	selfVecOut(595) =                            self.xDelay.h( 2, 1);
	selfVecOut(596) =                            self.xDelay.h( 2, 2);
	selfVecOut(597) =                            self.xDelay.h( 2, 3);
	selfVecOut(598) =                            self.xDelay.h( 2, 4);
	selfVecOut(599) =                            self.xDelay.h( 2, 5);
	selfVecOut(600) =                            self.xDelay.h( 2, 6);
	selfVecOut(601) =                            self.xDelay.h( 2, 7);
	selfVecOut(602) =                            self.xDelay.h( 2, 8);
	selfVecOut(603) =                            self.xDelay.h( 2, 9);
	selfVecOut(604) =                            self.xDelay.h( 2,10);
	selfVecOut(605) =                            self.xDelay.h( 3, 1);
	selfVecOut(606) =                            self.xDelay.h( 3, 2);
	selfVecOut(607) =                            self.xDelay.h( 3, 3);
	selfVecOut(608) =                            self.xDelay.h( 3, 4);
	selfVecOut(609) =                            self.xDelay.h( 3, 5);
	selfVecOut(610) =                            self.xDelay.h( 3, 6);
	selfVecOut(611) =                            self.xDelay.h( 3, 7);
	selfVecOut(612) =                            self.xDelay.h( 3, 8);
	selfVecOut(613) =                            self.xDelay.h( 3, 9);
	selfVecOut(614) =                            self.xDelay.h( 3,10);
	selfVecOut(615) =                            self.xDelay.h( 4, 1);
	selfVecOut(616) =                            self.xDelay.h( 4, 2);
	selfVecOut(617) =                            self.xDelay.h( 4, 3);
	selfVecOut(618) =                            self.xDelay.h( 4, 4);
	selfVecOut(619) =                            self.xDelay.h( 4, 5);
	selfVecOut(620) =                            self.xDelay.h( 4, 6);
	selfVecOut(621) =                            self.xDelay.h( 4, 7);
	selfVecOut(622) =                            self.xDelay.h( 4, 8);
	selfVecOut(623) =                            self.xDelay.h( 4, 9);
	selfVecOut(624) =                            self.xDelay.h( 4,10);
	selfVecOut(625) =                            self.xDelay.h( 5, 1);
	selfVecOut(626) =                            self.xDelay.h( 5, 2);
	selfVecOut(627) =                            self.xDelay.h( 5, 3);
	selfVecOut(628) =                            self.xDelay.h( 5, 4);
	selfVecOut(629) =                            self.xDelay.h( 5, 5);
	selfVecOut(630) =                            self.xDelay.h( 5, 6);
	selfVecOut(631) =                            self.xDelay.h( 5, 7);
	selfVecOut(632) =                            self.xDelay.h( 5, 8);
	selfVecOut(633) =                            self.xDelay.h( 5, 9);
	selfVecOut(634) =                            self.xDelay.h( 5,10);
	selfVecOut(635) =                            self.xDelay.h( 6, 1);
	selfVecOut(636) =                            self.xDelay.h( 6, 2);
	selfVecOut(637) =                            self.xDelay.h( 6, 3);
	selfVecOut(638) =                            self.xDelay.h( 6, 4);
	selfVecOut(639) =                            self.xDelay.h( 6, 5);
	selfVecOut(640) =                            self.xDelay.h( 6, 6);
	selfVecOut(641) =                            self.xDelay.h( 6, 7);
	selfVecOut(642) =                            self.xDelay.h( 6, 8);
	selfVecOut(643) =                            self.xDelay.h( 6, 9);
	selfVecOut(644) =                            self.xDelay.h( 6,10);
	selfVecOut(645) =                            self.xDelay.h( 7, 1);
	selfVecOut(646) =                            self.xDelay.h( 7, 2);
	selfVecOut(647) =                            self.xDelay.h( 7, 3);
	selfVecOut(648) =                            self.xDelay.h( 7, 4);
	selfVecOut(649) =                            self.xDelay.h( 7, 5);
	selfVecOut(650) =                            self.xDelay.h( 7, 6);
	selfVecOut(651) =                            self.xDelay.h( 7, 7);
	selfVecOut(652) =                            self.xDelay.h( 7, 8);
	selfVecOut(653) =                            self.xDelay.h( 7, 9);
	selfVecOut(654) =                            self.xDelay.h( 7,10);
	selfVecOut(655) =                            self.xDelay.h( 8, 1);
	selfVecOut(656) =                            self.xDelay.h( 8, 2);
	selfVecOut(657) =                            self.xDelay.h( 8, 3);
	selfVecOut(658) =                            self.xDelay.h( 8, 4);
	selfVecOut(659) =                            self.xDelay.h( 8, 5);
	selfVecOut(660) =                            self.xDelay.h( 8, 6);
	selfVecOut(661) =                            self.xDelay.h( 8, 7);
	selfVecOut(662) =                            self.xDelay.h( 8, 8);
	selfVecOut(663) =                            self.xDelay.h( 8, 9);
	selfVecOut(664) =                            self.xDelay.h( 8,10);
	selfVecOut(665) =                            self.xDelay.h( 9, 1);
	selfVecOut(666) =                            self.xDelay.h( 9, 2);
	selfVecOut(667) =                            self.xDelay.h( 9, 3);
	selfVecOut(668) =                            self.xDelay.h( 9, 4);
	selfVecOut(669) =                            self.xDelay.h( 9, 5);
	selfVecOut(670) =                            self.xDelay.h( 9, 6);
	selfVecOut(671) =                            self.xDelay.h( 9, 7);
	selfVecOut(672) =                            self.xDelay.h( 9, 8);
	selfVecOut(673) =                            self.xDelay.h( 9, 9);
	selfVecOut(674) =                            self.xDelay.h( 9,10);
	selfVecOut(675) =                            self.xDelay.h(10, 1);
	selfVecOut(676) =                            self.xDelay.h(10, 2);
	selfVecOut(677) =                            self.xDelay.h(10, 3);
	selfVecOut(678) =                            self.xDelay.h(10, 4);
	selfVecOut(679) =                            self.xDelay.h(10, 5);
	selfVecOut(680) =                            self.xDelay.h(10, 6);
	selfVecOut(681) =                            self.xDelay.h(10, 7);
	selfVecOut(682) =                            self.xDelay.h(10, 8);
	selfVecOut(683) =                            self.xDelay.h(10, 9);
	selfVecOut(684) =                            self.xDelay.h(10,10);
	selfVecOut(685) =                        self.xDelay.delay( 1, 1);
	selfVecOut(686) =                        self.xDelay.index( 1, 1);
	selfVecOut(687) =                         self.xLowPass.dt( 1, 1);
	selfVecOut(688) =                       self.xLowPass.fcut( 1, 1);
	selfVecOut(689) =                      self.xLowPass.state( 1, 1);
	selfVecOut(690) =                      self.xLowPass.state( 2, 1);
	selfVecOut(691) =                      self.xLowPass.state( 3, 1);
	selfVecOut(692) =                      self.xLowPass.state( 4, 1);
	selfVecOut(693) =                      self.xLowPass.state( 5, 1);
	selfVecOut(694) =                      self.xLowPass.state( 6, 1);
	selfVecOut(695) =                      self.xLowPass.state( 7, 1);
	selfVecOut(696) =                      self.xLowPass.state( 8, 1);
	selfVecOut(697) =                      self.xLowPass.state( 9, 1);
	selfVecOut(698) =                      self.xLowPass.state(10, 1);
	selfVecOut(699) =                        self.z_pub_thresh( 1, 1);
end

function self = LocalPositionEstimator( self, timestamp, dt )

% 	% required standard deviation of estimate for estimator to publish data
% 	% UINT32
% 	self.EST_STDDEV_XY_VALID = 2.0; % 2.0 m
% 	self.EST_STDDEV_Z_VALID = 2.0; % 2.0 m
% 	self.EST_STDDEV_TZ_VALID = 2.0; % 2.0 m
% 
% 	% float
% 	self.P_MAX = 1.0e6; % max allowed value in state covariance
% 	self.LAND_RATE = 10.0; % rate of land detector correction
% 
% 	% char
% 	% self.msg_label = '(lpe) ';  % rate of land detector correction
% 
% 	self.EST_XY = uint8(2^0);
% 	self.EST_Z  = uint8(2^1);
% 	self.EST_TZ = uint8(2^2);
% 
% 	self.BIAS_MAX = 1e-1;
% 
% 	self.FUSE_GPS            = uint8(2^0);
% 	self.FUSE_FLOW           = uint8(2^1);
% 	self.FUSE_VIS_POS        = uint8(2^2);
% 	self.FUSE_VIS_YAW        = uint8(2^3);
% 	self.FUSE_LAND           = uint8(2^4);
% 	self.FUSE_PUB_AGL_Z      = uint8(2^5);
% 	self.FUSE_FLOW_GYRO_COMP = uint8(2^6);
% 	self.FUSE_BARO           = uint8(2^7);
% 
% 	self.SENSOR_BARO   = uint8(2^0);
% 	self.SENSOR_GPS    = uint8(2^1);
% 	self.SENSOR_LIDAR  = uint8(2^2);
% 	self.SENSOR_FLOW   = uint8(2^3);
% 	self.SENSOR_SONAR  = uint8(2^4);
% 	self.SENSOR_VISION = uint8(2^5);
% 	self.SENSOR_MOCAP  = uint8(2^6);
% 	self.SENSOR_LAND   = uint8(2^7);
% 
% 	self.BETA_TABLE = [ 0, ...
% 				        8.82050518214, ...
% 				        12.094592431,  ...
% 				        13.9876612368, ...
% 				        16.0875642296, ...
% 				        17.8797700658, ...
% 				        19.6465647819 ];
                    
    if (~self.initialized)
        self = BlockLocalPositionEstimator( self );
        self.initialized = 1;
        self = initialize_blocks( dt, self ); % FIX THIS
    end

    % Run LPE
    self = update( self, timestamp );
    
end

% #include "BlockLocalPositionEstimator.hpp"
% #include <drivers/drv_hrt.h>
% #include <systemlib/mavlink_log.h>
% #include <fcntl.h>
% #include <systemlib/err.h>
% #include <matrix/math.hpp>
% #include <cstdlib>

% orb_advert_t mavlink_log_pub = nullptr;

% NEED TO TAKE CARE OF INITIALIZATION
% BlockLocalPositionEstimator::
function self = BlockLocalPositionEstimator( self )
	%% START
	% % this block has no parent, and has name LPE
	% SuperBlock(nullptr, "LPE"),
	% % subscriptions, set rate, add to list
	% self.sub_armed(ORB_ID(actuator_armed), 1000 / 2, 0, &getSubscriptions()),
	% self.sub_land(ORB_ID(vehicle_land_detected), 1000 / 2, 0, &getSubscriptions()),
	% self.sub_att(ORB_ID(vehicle_attitude), 1000 / 100, 0, &getSubscriptions()),
	% % set flow max update rate higher than expected to we don't lose packets
	% self.sub_flow(ORB_ID(optical_flow), 1000 / 100, 0, &getSubscriptions()),
	% % main prediction loop, 100 hz
	% self.sub_sensor(ORB_ID(sensor_combined), 1000 / 100, 0, &getSubscriptions()),
	% % status updates 2 hz
	% self.sub_param_update(ORB_ID(parameter_update), 1000 / 2, 0, &getSubscriptions()),
	% self.sub_manual(ORB_ID(manual_control_setpoint), 1000 / 2, 0, &getSubscriptions()),
	% % gps 10 hz
	% self.sub_gps(ORB_ID(vehicle_gps_position), 1000 / 10, 0, &getSubscriptions()),
	% % vision 50 hz
	% self.sub_vision_pos(ORB_ID(vehicle_vision_position), 1000 / 50, 0, &getSubscriptions()),
	% % mocap 50 hz
	% self.sub_mocap(ORB_ID(att_pos_mocap), 1000 / 50, 0, &getSubscriptions()),
	% % all distance sensors, 10 hz
	% self.sub_dist0(ORB_ID(distance_sensor), 1000 / 10, 0, &getSubscriptions()),
	% self.sub_dist1(ORB_ID(distance_sensor), 1000 / 10, 1, &getSubscriptions()),
	% self.sub_dist2(ORB_ID(distance_sensor), 1000 / 10, 2, &getSubscriptions()),
	% self.sub_dist3(ORB_ID(distance_sensor), 1000 / 10, 3, &getSubscriptions()),
	% self.dist_subs(),
	% self.sub_lidar(nullptr),
	% self.sub_sonar(nullptr),

	% % publications
	% self.pub_lpos(ORB_ID(vehicle_local_position), -1, &getPublications()),
	% self.pub_gpos(ORB_ID(vehicle_global_position), -1, &getPublications()),
	% self.pub_est_status(ORB_ID(estimator_status), -1, &getPublications()),
	% self.pub_innov(ORB_ID(ekf2_innovations), -1, &getPublications()),

	% % map projection
	% self.map_ref(),

	% % block parameters
	% self.fusion(this, "FUSION"),
	% self.vxy_pub_thresh(this, "VXY_PUB"),
	% self.z_pub_thresh(this, "Z_PUB"),
	% self.sonar_z_stddev(this, "SNR_Z"),
	% self.sonar_z_offset(this, "SNR_OFF_Z"),
	% self.lidar_z_stddev(this, "LDR_Z"),
	% self.lidar_z_offset(this, "LDR_OFF_Z"),
	% self.accel_xy_stddev(this, "ACC_XY"),
	% self.accel_z_stddev(this, "ACC_Z"),
	% self.baro_stddev(this, "BAR_Z"),
	% self.gps_delay(this, "GPS_DELAY"),
	% self.gps_xy_stddev(this, "GPS_XY"),
	% self.gps_z_stddev(this, "GPS_Z"),
	% self.gps_vxy_stddev(this, "GPS_VXY"),
	% self.gps_vz_stddev(this, "GPS_VZ"),
	% self.gps_eph_max(this, "EPH_MAX"),
	% self.gps_epv_max(this, "EPV_MAX"),
	% self.vision_xy_stddev(this, "VIS_XY"),
	% self.vision_z_stddev(this, "VIS_Z"),
	% self.vision_delay(this, "VIS_DELAY"),
	% self.mocap_p_stddev(this, "VIC_P"),
	% self.flow_z_offset(this, "FLW_OFF_Z"),
	% self.flow_scale(this, "FLW_SCALE"),
	% %_flow_board_x_offs(NULL, "SENS_FLW_XOFF"),
	% %_flow_board_y_offs(NULL, "SENS_FLW_YOFF"),
	% self.flow_min_q(this, "FLW_QMIN"),
	% self.flow_r(this, "FLW_R"),
	% self.flow_rr(this, "FLW_RR"),
	% self.land_z_stddev(this, "LAND_Z"),
	% self.land_vxy_stddev(this, "LAND_VXY"),
	% self.pn_p_noise_density(this, "PN_P"),
	% self.pn_v_noise_density(this, "PN_V"),
	% self.pn_b_noise_density(this, "PN_B"),
	% self.pn_t_noise_density(this, "PN_T"),
	% self.t_max_grade(this, "T_MAX_GRADE"),

	% % init origin
	% self.fake_origin(this, "FAKE_ORIGIN"),
	% self.init_origin_lat(this, "LAT"),
	% self.init_origin_lon(this, "LON"),

	% % flow gyro
	% self.flow_gyro_x_high_pass(this, "FGYRO_HP"),
	% self.flow_gyro_y_high_pass(this, "FGYRO_HP"),

	% % stats
	% self.baroStats(this, ""),
	% self.sonarStats(this, ""),
	% self.lidarStats(this, ""),
	% self.flowQStats(this, ""),
	% self.visionStats(this, ""),
	% self.mocapStats(this, ""),
	% self.gpsStats(this, ""),

	% % low pass
	% self.xLowPass(this, "X_LP"),
	% % use same lp constant for agl
	% self.aglLowPass(this, "X_LP"),

	% % delay
	% self.xDelay(this, ""),
	% self.tDelay(this, ""),

	% % misc
	% self.polls(),
	% self.timeStamp(hrt_absolute_time()),
	% self.time_origin(0),
	% self.timeStampLastBaro(hrt_absolute_time()),
	% self.time_last_hist(0),
	% self.time_last_flow(0),
	% self.time_last_baro(0),
	% self.time_last_gps(0),
	% self.time_last_lidar(0),
	% self.time_last_sonar(0),
	% self.time_init_sonar(0),
	% self.time_last_vision_p(0),
	% self.time_last_mocap(0),
	% self.time_last_land(0),

	% % reference altitudes
	% self.altOrigin(0),
	% self.altOriginInitialized(0),
	% self.baroAltOrigin(0),
	% self.gpsAltOrigin(0),

	% % status
	% self.receivedGps(0),
	% self.lastArmedState(0),

	% % masks
	% self.sensorTimeout(255),
	% self.sensorFault(0),
	% self.estimatorInitialized(0)
	%% INIT END

	% assign distance subs to array
% 	self.dist_subs(0) = self.sub_dist0;
% 	self.dist_subs(1) = self.sub_dist1;
% 	self.dist_subs(2) = self.sub_dist2;
% 	self.dist_subs(3) = self.sub_dist3;

	% setup event triggering based on new flow messages to integrate
	% self.polls(POLL_FLOW).fd = self.sub_flow.getHandle();
	% self.polls(POLL_FLOW).events = POLLIN;

	% self.polls(POLL_PARAM).fd = self.sub_param_update.getHandle();
	% self.polls(POLL_PARAM).events = POLLIN;

	% self.polls(POLL_SENSORS).fd = self.sub_sensor.getHandle();
	% self.polls(POLL_SENSORS).events = POLLIN;

	% initialize A, B,  P, x, u
	n_x = 10; n_u = 3;
	self.x = zeros(n_x, 1);%.setZero();
	self.u = zeros(n_u,1);
	self = initSS( self );

	% map
	self.map_ref.init_done = 0;

	% intialize parameter dependent matrices
	% self = updateParams( self ); - not needed since we assign everything
	% above

	% print fusion settings to console
	% printf(( ['(lpe) fuse gps: %d, flow: %d, vis_pos: %d, ' ...
	%        'vis_yaw: %d, land: %d, pub_agl_z: %d, flow_gyro: %d\n'] ), ...
	%        bitand( self.fusion, self.FUSE_GPS)             ~= 0, ...
	%        bitand( self.fusion, self.FUSE_FLOW )           ~= 0, ...
	%        bitand( self.fusion, self.FUSE_VIS_POS )        ~= 0, ...
	%        bitand( self.fusion, self.FUSE_VIS_YAW )        ~= 0, ...
	%        bitand( self.fusion, self.FUSE_LAND )           ~= 0, ...
	%        bitand( self.fusion, self.FUSE_PUB_AGL_Z )      ~= 0, ...
	%        bitand( self.fusion, self.FUSE_FLOW_GYRO_COMP ) ~= 0 );
end

% BlockLocalPositionEstimator::~BlockLocalPositionEstimator()
% {
% }

%Vector<float, BlockLocalPositionEstimator::n_x> BlockLocalPositionEstimator::
%float t
%const Vector<float, BlockLocalPositionEstimator::n_x> &x
%const Vector<float, BlockLocalPositionEstimator::n_u> &u
function output = dynamics( ~, x, u, A, B )
	output = A * x + B * u;
end

% Add all commented out sensors
% self.pub_innov.update( self );
% void BlockLocalPositionEstimator::
function self = update( self, timestamp )
%UPDATE
    X_x = 1; X_y = 2; X_z = 3; X_vx = 4; X_vy = 5; X_vz = 6;
	X_bx = 7; X_by = 8; X_bz = 9; X_tz = 10; n_x = 10;
	% Probably bypass all this stuff
	% wait for a sensor update, check for exit condition every 100 ms int
	% ret = px4_poll(self.polls, 3, 100);

	% if (ret < 0)
	% 	return;
	% end

	%uint64_t
	newTimeStamp = timestamp;
	%float
	dt = (newTimeStamp - self.timeStamp) / 1.0e6;
	self.timeStamp = newTimeStamp;

	% set dt for all child blocks
	self = setDt( dt, self );

	% auto-detect connected rangefinders while not armed bool - maybe bypass?
	armedState = self.sub_armed.armed;

    % Probably not needed
% 	if (~armedState && (self.sub_lidar == nullptr || self.sub_sonar == nullptr))
% 
% 		% detect distance sensors
% 		for i = 1:DIST_SUBS %i < N_DIST_SUBS; i++)
% 			%uORB::Subscription<distance_sensor_s> *s = self.dist_subs(i);
% 			s = self.dist_subs(i);
% 
% 			if (s == self.sub_lidar || s == self.sub_sonar)
% 				continue;
% 			end
% 
% 			if ( s.updated )
% 				s.update();
% 
% 				if (s.timestamp == 0)
% 					continue;
% 				end
% 
% 				if (s.type == MAV_DISTANCE_SENSOR_LASER && ...
% 				    self.sub_lidar == nullptr)
% 					self.sub_lidar = s;
% 					% mavlink_and_console_log_info(&mavlink_log_pub, '%sLidar detected with ID %i', self.msg_label, i);
%                 elseif (s.type == MAV_DISTANCE_SENSOR_ULTRASOUND && ...
% 					   self.sub_sonar == nullptr)
% 					self.sub_sonar = s;
% 					% mavlink_and_console_log_info(&mavlink_log_pub, '%sSonar detected with ID %i', self.msg_label, i);
% 				end
% 			end
% 		end
% 	end

	% reset pos, vel, and terrain on arming

	% XXX this will be re-enabled for indoor use cases using a
	% selection param, but is really not helping outdoors
	% right now.

	% if (~self.lastArmedState && armedState) {

	% 	% we just armed, we are at origin on the ground
	% 	self.x(X_x) = 0;
	% 	self.x(X_y) = 0;
	% 	% reset Z or not? self.x(X_z) = 0;

	% 	% we aren't moving, all velocities are zero
	% 	self.x(X_vx) = 0;
	% 	self.x(X_vy) = 0;
	% 	self.x(X_vz) = 0;

	% 	% assume we are on the ground, so terrain alt is local alt
	% 	self.x(X_tz) = self.x(X_z);

	% 	% reset lowpass filter as well
	% 	self.xLowPass.setState(self.x);
	% 	self.aglLowPass.setState(0);
	% }

	self.lastArmedState = armedState;

	% see which updates are available all bool
	paramsUpdated = self.sub_param_update.updated;
	baroUpdated = 0;

	if ( bitand(self.fusion, self.FUSE_BARO) && self.sub_sensor.updated )
		% int32_t
		baro_timestamp_relative = self.sub_sensor.baro_timestamp_relative;

		if ( baro_timestamp_relative ~= self.sub_sensor.RELATIVE_TIMESTAMP_INVALID )
			% uint64_t 
			baro_timestamp = self.sub_sensor.timestamp + ...
						  self.sub_sensor.baro_timestamp_relative;

			if (baro_timestamp ~= self.timeStampLastBaro)
				baroUpdated = 1;
				self.timeStampLastBaro = baro_timestamp;
			end
		end
	end

	% All bool
	flowUpdated   = bitand(self.fusion, self.FUSE_FLOW) && self.sub_flow.updated;
	gpsUpdated    = bitand(self.fusion, self.FUSE_GPS) && self.sub_gps.updated;
	visionUpdated = bitand(self.fusion, self.FUSE_VIS_POS) && self.sub_vision_pos.updated;
	mocapUpdated  = self.sub_mocap.updated;
	lidarUpdated  = self.sub_lidar.present && self.sub_lidar.updated;
	sonarUpdated  = self.sub_sonar.present && self.sub_sonar.updated;
	landUpdated   = landed( self ) ...
			   && ((self.timeStamp - self.time_last_land) > (1.0e6 / self.LAND_RATE)); % throttle rate

	% get new data - maybe not necessary
	% self = updateSubscriptions( self );

	% update parameters
	if ( paramsUpdated )
		%self = updateParams( self );
		self = updateSSParams( self );
	end

	% is xy valid? bool
	vxy_stddev_ok = 0;

	if (max(self.P(X_vx, X_vx), self.P(X_vy, X_vy)) < (self.vxy_pub_thresh * self.vxy_pub_thresh))
		vxy_stddev_ok = 1;
	end

	if bitand(self.estimatorInitialized, self.EST_XY)
		% if valid and gps has timed out, set to not valid
		if (~vxy_stddev_ok && bitand(self.sensorTimeout, self.SENSOR_GPS))
			self.estimatorInitialized = bitand(self.estimatorInitialized, bitcmp( self.EST_XY , 'uint8' ));
		end
	else
		if (vxy_stddev_ok)
			if (   ~bitand(self.sensorTimeout, self.SENSOR_GPS)       ...
			    || ~bitand(self.sensorTimeout, self.SENSOR_FLOW)   ...
			    || ~bitand(self.sensorTimeout, self.SENSOR_VISION) ...
			    || ~bitand(self.sensorTimeout, self.SENSOR_MOCAP)  ...
			    || ~bitand(self.sensorTimeout, self.SENSOR_LAND)   ...
			   )
				self.estimatorInitialized = bitor( self.estimatorInitialized, self.EST_XY );
			end
		end
	end

	% is z valid? bool
	z_stddev_ok = sqrt(self.P(X_z, X_z)) < self.z_pub_thresh;

	if bitand(self.estimatorInitialized, self.EST_Z)
		% if valid and baro has timed out, set to not valid
		if (~z_stddev_ok && bitand(self.sensorTimeout, self.SENSOR_BARO))
			self.estimatorInitialized = bitand(self.estimatorInitialized, bitcmp( self.EST_Z, 'uint8' ));
		end

	else
		if (z_stddev_ok)
			self.estimatorInitialized = bitor( self.estimatorInitialized, self.EST_Z );
		end
	end

	% is terrain valid?
	tz_stddev_ok = sqrt(self.P(X_tz, X_tz)) < self.z_pub_thresh;

	if bitand(self.estimatorInitialized, self.EST_TZ)
		if (~tz_stddev_ok)
			self.estimatorInitialized = bitand(self.estimatorInitialized, bitcmp( self.EST_TZ, 'uint8' ));
		end

	else
		if (tz_stddev_ok)
			self.estimatorInitialized = bitor( self.estimatorInitialized, self.EST_TZ );
		end
	end

	% check timeouts
	self = checkTimeouts( self );

	% if we have no lat, lon initialize projection to LPE_LAT, LPE_LON parameters
	if (~self.map_ref.init_done && bitand(self.estimatorInitialized, self.EST_XY) && self.fake_origin)
		[~, self.map_ref] = map_projection_init_timestamped(self.map_ref, ...
				    self.init_origin_lat, ...
				    self.init_origin_lon, self.timeStamp);

		% set timestamp when origin was set to current time
		self.time_origin = self.timeStamp;

% 		mavlink_and_console_log_info(mavlink_log_pub, '(lpe) global origin init (parameter) : lat %6.2f lon %6.2f alt %5.1f m', ...
% 					     double(self.init_origin_lat), double(self.init_origin_lon), double(self.altOrigin));

	end

	% reinitialize x if necessary bool
	reinit_x = 0;

	for i = 1:n_x %; i < n_x; i++)
		% should we do a reinit
		% of sensors here?
		% don't want it to take too long
		if (~isfinite(self.x(i)))
			reinit_x = 1;
			% mavlink_and_console_log_info(mavlink_log_pub, '%sreinit x, x(%d) not finite', self.msg_label, i);
			break;
		end
	end

	if (reinit_x)
		for i = 1:n_x %; i < n_x; i++)
			self.x(i) = 0;
		end

		% mavlink_and_console_log_info(mavlink_log_pub, '%sreinit x', self.msg_label);
	end

	% force P symmetry and reinitialize P if necessary bool
	reinit_P = 0;

	for i = 1:n_x %; i < n_x; i++)
		for j = 1:i %; j <= i; j++)
			if (~isfinite(self.P(i, j)))
% 				mavlink_and_console_log_info(mavlink_log_pub, ...
% 							     '%sreinit P (%d, %d) not finite', self.msg_label, i, j);
				reinit_P = 1;
			end

			if (i == j)
				% make sure diagonal elements are positive
				if (self.P(i, i) <= 0)
% 					mavlink_and_console_log_info(&mavlink_log_pub, ...
% 								     '%sreinit P (%d, %d) negative', self.msg_label, i, j);
					reinit_P = 1;
				end
			else
				% copy elememnt from upper triangle to force
				% symmetry
				self.P(j, i) = self.P(i, j);
			end

			if (reinit_P)
				break;
			end
		end

		if (reinit_P)
			break;
		end
	end

	if (reinit_P)
		self = initP( self );
	end

	% do prediction
	self = predict( self );

	% sensor corrections/ initializations
% 	if (gpsUpdated)
% 		if bitand( self.sensorTimeout, self.SENSOR_GPS )
% 			self = gpsInit( self );
% 		else
% 			self = gpsCorrect( self );
% 		end
% 	end

	if (baroUpdated)
		if bitand( self.sensorTimeout, self.SENSOR_BARO )
			self = baroInit( self );
		else
			self = baroCorrect( self );
		end
	end

% 	if (lidarUpdated)
% 		if bitand( self.sensorTimeout, self.SENSOR_LIDAR )
% 			self = lidarInit( self );
% 		else
% 			self = lidarCorrect( self );
% 		end
% 	end
% 
% 	if (sonarUpdated)
% 		if bitand( self.sensorTimeout, self.SENSOR_SONAR )
% 			self = sonarInit( self );
% 		else
% 			self = sonarCorrect( self );
% 		end
% 	end
% 
% 	if (flowUpdated)
% 		if bitand( self.sensorTimeout, self.SENSOR_FLOW )
% 			self = flowInit( self );
% 		else
% 			self = flowCorrect( self );
% 		end
% 	end
% 
% 	if (visionUpdated)
% 		if bitand( self.sensorTimeout, self.SENSOR_VISION )
% 			self = visionInit( self );
% 		else
% 			self = visionCorrect( self );
% 		end
% 	end

	if (mocapUpdated)
		if bitand( self.sensorTimeout, self.SENSOR_MOCAP )
			self = mocapInit( self );
		else
			self = mocapCorrect( self );
		end
	end

	if (landUpdated)
		if bitand( self.sensorTimeout, self.SENSOR_LAND )
			self = landInit( self );
		else
			self = landCorrect( self );
		end
	end

	if (self.altOriginInitialized)
		% update all publications if possible
		self = publishLocalPos( self );
		self = publishEstimatorStatus( self );
		% self.pub_innov.update( self );

		if ( bitand(self.estimatorInitialized, self.EST_XY) && (self.map_ref.init_done || self.fake_origin))
			self = publishGlobalPos( self );
		end
	end

	% propagate delayed state, no matter what
	% if state is frozen, delayed state still
	% needs to be propagated with frozen state
	dt_hist = 1.0e-6 * (self.timeStamp - self.time_last_hist);

	if ( (self.time_last_hist == 0) || (dt_hist > self.HIST_STEP) )
		[~, self.tDelay] = updateBlockDelay( self.tDelay, self.timeStamp );
		[~, self.xDelay] = updateBlockDelay( self.xDelay, self.x );
		self.time_last_hist = self.timeStamp;
	end
end

% Add all commented out functions
%void BlockLocalPositionEstimator::
function self = checkTimeouts( self )
%CHECKTIMEOUTS Check sensor timeouts
	self = baroCheckTimeout( self );
% 	self = gpsCheckTimeout( self );
% 	self = lidarCheckTimeout( self );
% 	self = flowCheckTimeout( self );
% 	self = sonarCheckTimeout( self );
% 	self = visionCheckTimeout( self );
	self = mocapCheckTimeout( self );
	self = landCheckTimeout( self );
end

% bool BlockLocalPositionEstimator::
function output = landed( self )
%LANDED
	if (~bitand(self.fusion, self.FUSE_LAND))
		% return 0;
		output = 0;
		return;
	end

	disarmed_not_falling = (~self.sub_armed.armed) && (~self.sub_land.freefall);

	output = double( self.sub_land.landed || disarmed_not_falling );
end

% void BlockLocalPositionEstimator::
function self = publishLocalPos( self )
%PUBLISHLOCALPOS
	X_x = 1; X_y = 2; X_z = 3; X_vx = 4; X_vy = 5; X_vz = 6;
	X_bx = 7; X_by = 8; X_bz = 9; X_tz = 10; n_x = 10;

	%const Vector<float, n_x> &
	xLP = self.xLowPass.state;

	% lie about eph/epv to allow visual odometry only navigation when velocity est. good
	% All float
	vxy_stddev = sqrt(self.P(X_vx, X_vx) + self.P(X_vy, X_vy));
	epv = sqrt(self.P(X_z, X_z));
	eph = sqrt(self.P(X_x, X_x) + self.P(X_y, X_y));
	eph_thresh = 3.0;
	epv_thresh = 3.0;

	if (vxy_stddev < self.vxy_pub_thresh)
		if (eph > eph_thresh)
			eph = eph_thresh;
		end

		if (epv > epv_thresh)
			epv = epv_thresh;
		end
	end

	% publish local position
	if (isfinite(self.x(X_x)) && isfinite(self.x(X_y)) && isfinite(self.x(X_z)) && ...
	    isfinite(self.x(X_vx)) && isfinite(self.x(X_vy)) ...
	    && isfinite(self.x(X_vz)))
		self.pub_lpos.timestamp  = self.timeStamp;
		self.pub_lpos.xy_valid   = double( bitand( self.estimatorInitialized, self.EST_XY ));
		self.pub_lpos.z_valid    = double( bitand( self.estimatorInitialized, self.EST_Z ));
		self.pub_lpos.v_xy_valid = double( bitand( self.estimatorInitialized, self.EST_XY ));
		self.pub_lpos.v_z_valid  = double( bitand( self.estimatorInitialized, self.EST_Z ));
		self.pub_lpos.x = xLP(X_x); 	% north
		self.pub_lpos.y = xLP(X_y);  	% east

		if bitand(self.fusion, self.FUSE_PUB_AGL_Z)
			self.pub_lpos.z = -self.aglLowPass.state; % agl

		else
			self.pub_lpos.z = xLP(X_z); 	% down
		end

		self.pub_lpos.vx = xLP(X_vx); % north
		self.pub_lpos.vy = xLP(X_vy); % east
		self.pub_lpos.vz = xLP(X_vz); % down

		% this estimator does not provide a separate vertical position time derivative estimate, so use the vertical velocity
		self.pub_lpos.z_deriv = xLP(X_vz);

		self.pub_lpos.yaw = self.eul(3);
		self.pub_lpos.xy_global = double( bitand(self.estimatorInitialized, self.EST_XY));
		self.pub_lpos.z_global = double( ~bitand(self.sensorTimeout, self.SENSOR_BARO));
		self.pub_lpos.ref_timestamp = self.time_origin;
		self.pub_lpos.ref_lat = self.map_ref.lat_rad * 180 / pi;
		self.pub_lpos.ref_lon = self.map_ref.lon_rad * 180 / pi;
		self.pub_lpos.ref_alt = self.altOrigin;
		self.pub_lpos.dist_bottom = self.aglLowPass.state;
		self.pub_lpos.dist_bottom_rate = - xLP(X_vz);
		self.pub_lpos.surface_bottom_timestamp = self.timeStamp;
		% we estimate agl even when we don't have terrain info
		% if you are in terrain following mode this is important
		% so that if terrain estimation fails there isn't a
		% sudden altitude jump
		self.pub_lpos.dist_bottom_valid = double( bitand(self.estimatorInitialized, self.EST_Z));
		self.pub_lpos.eph = eph;
		self.pub_lpos.epv = epv;
		% self.pub_lpos.update();
		% TODO provide calculated values for these
		self.pub_lpos.evh = 0.0;
		self.pub_lpos.evv = 0.0;
	end
end

% void BlockLocalPositionEstimator::
function self = publishEstimatorStatus( self )
%PUBLISHESTIMATORSTATUS
	n_x = 10;
	self.pub_est_status.timestamp = self.timeStamp;

	for i = 1:n_x %; i < n_x; i++)
		self.pub_est_status.states(i) = self.x(i);
		self.pub_est_status.covariances(i) = self.P(i, i);
	end

	self.pub_est_status.n_states = n_x;
	self.pub_est_status.nan_flags = uint8( 0 );
	self.pub_est_status.health_flags = self.sensorFault;
	self.pub_est_status.timeout_flags = self.sensorTimeout;
	self.pub_est_status.pos_horiz_accuracy = self.pub_gpos.eph;
	self.pub_est_status.pos_vert_accuracy = self.pub_gpos.epv;

	% self.pub_est_status.update();
end

% void BlockLocalPositionEstimator::
function self = publishGlobalPos( self )
%PUBLISHGLOBALPOS
	X_x = 1; X_y = 2; X_z = 3; X_vx = 4; X_vy = 5; X_vz = 6;
	X_bx = 7; X_by = 8; X_bz = 9; X_tz = 10; n_x = 10;

	% publish global position double
	lat = 0;
	lon = 0;
	% const Vector<float, n_x> &
	xLP = self.xLowPass.state;
	[ ~, lat, lon ] = map_projection_reproject(self.map_ref, xLP(X_x), xLP(X_y), lat, lon);
	% float
	alt = -xLP(X_z) + self.altOrigin;

	% lie about eph/epv to allow visual odometry only navigation when velocity est. good all float
	vxy_stddev = sqrt(self.P(X_vx, X_vx) + self.P(X_vy, X_vy));
	epv = sqrt(self.P(X_z, X_z));
	eph = sqrt(self.P(X_x, X_x) + self.P(X_y, X_y));
	eph_thresh = 3.0;
	epv_thresh = 3.0;

	if (vxy_stddev < self.vxy_pub_thresh)
		if (eph > eph_thresh)
			eph = eph_thresh;
		end

		if (epv > epv_thresh)
			epv = epv_thresh;
		end
	end

	if (isfinite(lat) && isfinite(lon) && isfinite(alt) && ...
	    isfinite(xLP(X_vx)) && isfinite(xLP(X_vy)) && ...
	    isfinite(xLP(X_vz)))
		self.pub_gpos.timestamp = self.timeStamp;
		self.pub_gpos.time_utc_usec = self.sub_gps.time_utc_usec;
		self.pub_gpos.lat = lat;
		self.pub_gpos.lon = lon;
		self.pub_gpos.alt = alt;
		self.pub_gpos.vel_n = xLP(X_vx);
		self.pub_gpos.vel_e = xLP(X_vy);
		self.pub_gpos.vel_d = xLP(X_vz);

		% this estimator does not provide a separate vertical position time derivative estimate, so use the vertical velocity
		self.pub_gpos.pos_d_deriv = xLP(X_vz);

		self.pub_gpos.yaw = self.eul(3);
		self.pub_gpos.eph = eph;
		self.pub_gpos.epv = epv;
		self.pub_gpos.terrain_alt = self.altOrigin - xLP(X_tz);
		self.pub_gpos.terrain_alt_valid = double( bitand(self.estimatorInitialized, self.EST_TZ) );
		self.pub_gpos.dead_reckoning = double( ~bitand(self.estimatorInitialized, self.EST_XY) );
		self.pub_gpos.pressure_alt = self.sub_sensor.baro_alt_meter;
		% self.pub_gpos.update();
		% TODO provide calculated values for these
		self.pub_gpos.evh = 0.0;
		self.pub_gpos.evv = 0.0;
	end
end

% void BlockLocalPositionEstimator::
function self = initP( self )
%INIT_P Initialise P matrix

	X_x = 1; X_y = 2; X_z = 3; X_vx = 4; X_vy = 5; X_vz = 6;
	X_bx = 7; X_by = 8; X_bz = 9; X_tz = 10; n_x = 10;

	self.P = zeros( n_x, n_x );
	% initialize to twice valid condition
	self.P(X_x, X_x) = 2 * self.EST_STDDEV_XY_VALID * self.EST_STDDEV_XY_VALID;
	self.P(X_y, X_y) = 2 * self.EST_STDDEV_XY_VALID * self.EST_STDDEV_XY_VALID;
	self.P(X_z, X_z) = 2 * self.EST_STDDEV_Z_VALID * self.EST_STDDEV_Z_VALID;
	self.P(X_vx, X_vx) = 2 * self.vxy_pub_thresh * self.vxy_pub_thresh;
	self.P(X_vy, X_vy) = 2 * self.vxy_pub_thresh * self.vxy_pub_thresh;
	% use vxy thresh for vz init as well
	self.P(X_vz, X_vz) = 2 * self.vxy_pub_thresh * self.vxy_pub_thresh;
	% initialize bias uncertainty to small values to keep them stable
	self.P(X_bx, X_bx) = 1e-6;
	self.P(X_by, X_by) = 1e-6;
	self.P(X_bz, X_bz) = 1e-6;
	self.P(X_tz, X_tz) = 2 * self.EST_STDDEV_TZ_VALID * self.EST_STDDEV_TZ_VALID;
end

% DONE
%void BlockLocalPositionEstimator::
function self = initSS( self )
%INITSS Initialize state space model
	X_x = 1; X_y = 2; X_z = 3; X_vx = 4; X_vy = 5; X_vz = 6;
	X_bx = 7; X_by = 8; X_bz = 9; X_tz = 10; n_x = 10;
	U_ax = 1; U_ay = 2; U_az = 3; n_u = 3;

	self = initP( self );

	% dynamics matrix
	self.A = zeros(n_x, n_x);
	% derivative of position is velocity
	self.A(X_x, X_vx) = 1;
	self.A(X_y, X_vy) = 1;
	self.A(X_z, X_vz) = 1;

	% input matrix
	self.B = zeros(n_x, n_u);
	self.B(X_vx, U_ax) = 1;
	self.B(X_vy, U_ay) = 1;
	self.B(X_vz, U_az) = 1;

	% update components that depend on current state
	self = updateSSStates( self );
	self = updateSSParams( self );
end

%void BlockLocalPositionEstimator::
function self = updateSSStates( self )
%UPDATESSStates
	% derivative of velocity is accelerometer acceleration
	% (in input matrix) - bias (in body frame)
    X_x = 1; X_y = 2; X_z = 3; X_vx = 4; X_vy = 5; X_vz = 6;
	X_bx = 7; X_by = 8; X_bz = 9; X_tz = 10; n_x = 10;
	self.A(X_vx, X_bx) = -self.R_att(1, 1);
	self.A(X_vx, X_by) = -self.R_att(1, 2);
	self.A(X_vx, X_bz) = -self.R_att(1, 3);

	self.A(X_vy, X_bx) = -self.R_att(2, 1);
	self.A(X_vy, X_by) = -self.R_att(2, 2);
	self.A(X_vy, X_bz) = -self.R_att(2, 3);

	self.A(X_vz, X_bx) = -self.R_att(3, 1);
	self.A(X_vz, X_by) = -self.R_att(3, 2);
	self.A(X_vz, X_bz) = -self.R_att(3, 3);
end

%void BlockLocalPositionEstimator::
function self = updateSSParams( self )
%UPDATESSPARAMS Update steady state parameters
	
	% enum {X_x = 0, X_y, X_z, X_vx, X_vy, X_vz, X_bx, X_by, X_bz, X_tz, n_x};
	X_x = 1; X_y = 2; X_z = 3; X_vx = 4; X_vy = 5; X_vz = 6;
	X_bx = 7; X_by = 8; X_bz = 9; X_tz = 10; n_x = 10;

	% input noise covariance matrix
	self.R = zeros(3, 3); %.setZero();
	self.R(1, 1) = self.accel_xy_stddev * self.accel_xy_stddev;
	self.R(2, 2) = self.accel_xy_stddev * self.accel_xy_stddev;
	self.R(3, 3) = self.accel_z_stddev * self.accel_z_stddev;

	% process noise power matrix
	self.Q = zeros(n_x, n_x); %.setZero();
	%float
	pn_p_sq = self.pn_p_noise_density * self.pn_p_noise_density;
	%float
	pn_v_sq = self.pn_v_noise_density * self.pn_v_noise_density;
	self.Q(X_x, X_x) = pn_p_sq;
	self.Q(X_y, X_y) = pn_p_sq;
	self.Q(X_z, X_z) = pn_p_sq;
	self.Q(X_vx, X_vx) = pn_v_sq;
	self.Q(X_vy, X_vy) = pn_v_sq;
	self.Q(X_vz, X_vz) = pn_v_sq;

	% technically, the noise is in the body frame,
	% but the components are all the same, so
	% ignoring for now
	% float
	pn_b_sq = self.pn_b_noise_density * self.pn_b_noise_density;
	self.Q(X_bx, X_bx) = pn_b_sq;
	self.Q(X_by, X_by) = pn_b_sq;
	self.Q(X_bz, X_bz) = pn_b_sq;

	% terrain random walk noise ((m/s)/sqrt(hz)), scales with velocity
	%float
	pn_t_noise_density = ...
		self.pn_t_noise_density + ...
		(self.t_max_grade / 100.0) * ...
		sqrt(self.x(X_vx) * self.x(X_vx) + self.x(X_vy) * self.x(X_vy));
	self.Q(X_tz, X_tz) = pn_t_noise_density * pn_t_noise_density;
end

% void BlockLocalPositionEstimator::
function self = predict( self )
%PREDICT Prediction step
	% Definitions
	U_ax = 1; U_ay = 2; U_az = 3; n_u = 3;
	X_x = 1; X_y = 2; X_z = 3; X_vx = 4; X_vy = 5; X_vz = 6;
	X_bx = 7; X_by = 8; X_bz = 9; X_tz = 10; n_x = 10;

	% get acceleration
	q = self.sub_att.q; % matrix::Quaternion<float> q(&self.sub_att.get().q(0));
	self.eul = quat_to_euler( q ); %matrix::Euler<float>(q);
	self.R_att = quat_to_dcm( q ); % matrix::Dcm<float>(q);
	a = self.sub_sensor.accelerometer_m_s2; % Vector3f a(self.sub_sensor.get().accelerometer_m_s2);
	% note, bias is removed in dynamics function
	self.u = self.R_att * a;
	self.u(U_az) = self.u(U_az) + 9.81; % add g

	% update state space based on new states
	self = updateSSStates( self );

	% continuous time kalman filter prediction
	% integrate runge kutta 4th order
	% TODO move rk4 algorithm to matrixlib
	% https:%en.wikipedia.org/wiki/Runge%E2%80%93Kutta_methods
	h = self.dt; % float
	% Vector<float, n_x> k1, k2, k3, k4;
	k1 = zeros( n_x, 1 ); k2 = k1; k3 = k1; k4 = k1;
	k1 = dynamics(0, self.x, self.u, self.A, self.B);
	k2 = dynamics(h / 2, self.x + k1 * h / 2, self.u, self.A, self.B);
	k3 = dynamics(h / 2, self.x + k2 * h / 2, self.u, self.A, self.B);
	k4 = dynamics(h, self.x + k3 * h, self.u, self.A, self.B);
	
	% Vector<float, n_x>
	dx = (k1 + k2 * 2 + k3 * 2 + k4) * (h / 6);

	% don't integrate position if no valid xy data
	if ( ~( bitand( self.estimatorInitialized, self.EST_XY ) ) )
		dx(X_x) = 0;
		dx(X_vx) = 0;
		dx(X_y) = 0;
		dx(X_vy) = 0;
	end

	% don't integrate z if no valid z data
	if ( ~( bitand( self.estimatorInitialized, self.EST_Z) ) )
		dx(X_z) = 0;
	end

	% don't integrate tz if no valid tz data
	if ( ~( bitand( self.estimatorInitialized, self.EST_TZ ) ) )
		dx(X_tz) = 0;
	end

	% saturate bias all float
	bx = dx(X_bx) + self.x(X_bx);
	by = dx(X_by) + self.x(X_by);
	bz = dx(X_bz) + self.x(X_bz);

	if (abs(bx) > self.BIAS_MAX)
		bx = self.BIAS_MAX * bx / abs(bx);
		dx(X_bx) = bx - self.x(X_bx);
	end

	if (abs(by) > self.BIAS_MAX)
		by = self.BIAS_MAX * by / abs(by);
		dx(X_by) = by - self.x(X_by);
	end

	if (abs(bz) > self.BIAS_MAX)
		bz = self.BIAS_MAX * bz / abs(bz);
		dx(X_bz) = bz - self.x(X_bz);
	end

	% propagate
	self.x = self.x + dx;
	% Matrix<float, n_x, n_x>
	dP = (self.A * self.P + self.P * self.A' + ...
		self.B * self.R * self.B' + self.Q) * self.dt;

	% covariance propagation logic
	for i = 1:n_x %; i < n_x; i++)
		if (self.P(i, i) > self.P_MAX)
			% if diagonal element greater than max, stop propagating
			dP(i, i) = 0;

			for j = 1:n_x %; j < n_x; j++)
				dP(i, j) = 0;
				dP(j, i) = 0;
			end
		end
	end

	self.P = self.P + dP;
	[~, self.xLowPass] = block_lowpass_update( self.x, self.xLowPass );
	agl = self.x(X_tz) - self.x(X_z);
	[~, self.aglLowPass] = block_lowpass_update( agl, self.aglLowPass );
end

% Not examined - Probably not used
% int BlockLocalPositionEstimator::
function [ self, output, periods ] = getDelayPeriods( self, delay )
%GETDELAYPERIODS
	%float
	t_delay = 0;
	%uint8_t
	i_hist = 0;

	HIST_LEN = 10; % DELAY_MAX / HIST_STEP
	for i_hist = 2:HIST_LEN %; i_hist < HIST_LEN; i_hist++) {
		tmp = (self.timeStamp - self.tDelay(i_hist));
		t_delay = 1.0e-6 * tmp(1, 1);

		if (t_delay > delay)
			break;
		end
	end

	periods = i_hist;

	DELAY_MAX = 0.5;
	if (t_delay > DELAY_MAX)
		% mavlink_and_console_log_info(&mavlink_log_pub, '%sdelayed data old: %8.4f', self.msg_label, double(t_delay));
		output = 0;
		return;
	end

	output = 1;
end


%% ADDITIONAL FUNCTIONS

function out = quat_to_euler( data )
%QUAT_TO_EULER Create Euler angles vector from the quaternion
    out = [atan2(2.0 * (data(1) * data(2) + data(3) * data(4)), 1.0 - 2.0 * (data(2) * data(2) + data(3) * data(3)));
    asin(2.0 * (data(1) * data(3) - data(4) * data(2)));
    atan2(2.0 * (data(1) * data(4) + data(2) * data(3)), 1.0 - 2.0 * (data(3) * data(3) + data(4) * data(4)))];
end

function R  = quat_to_dcm( data )
%QUAT_TO_DCM Convert quaternion to DCM
%	From https:%github.com/PX4/Firmware/blob/master/src/lib/mathlib/math/Quaternion.hpp
    aSq = data(1) * data(1);
    bSq = data(2) * data(2);
    cSq = data(3) * data(3);
    dSq = data(4) * data(4);
    R = zeros(3,3);
    R(1,1) = aSq + bSq - cSq - dSq;
    R(1,2) = 2.0 * ( data(2) * data(3) - data(1) * data(4) );
    R(1,3) = 2.0 * ( data(1) * data(3) + data(2) * data(4) );
    R(2,1) = 2.0 * ( data(2) * data(3) + data(1) * data(4) );
    R(2,2) = aSq - bSq + cSq - dSq;
    R(2,3) = 2.0 * ( data(3) * data(4) - data(1) * data(2) );
    R(3,1) = 2.0 * ( data(2) * data(4) - data(1) * data(3) );
    R(3,2) = 2.0 * ( data(1) * data(2) + data(3) * data(4) );
    R(3,3) = aSq - bSq - cSq + dSq;
end

function [ out, lat, lon ] = map_projection_reproject( ref, x, y, lat, lon )
%MAP_PROJECTION_REPROJECT
    CONSTANTS_RADIUS_OF_EARTH = 6371000;
    M_PI = 3.14159265358979323846;
    
    if ( ~map_projection_initialized(ref))
        out = -1;
        return
    end

    x_rad = x / CONSTANTS_RADIUS_OF_EARTH;
    y_rad = y / CONSTANTS_RADIUS_OF_EARTH;
    c = sqrt(x_rad * x_rad + y_rad * y_rad);
    
    sin_c = sin(c);
    cos_c = cos(c);

    if (abs(c) > eps)
        lat_rad = asin(cos_c * ref.sin_lat + (x_rad * sin_c * ref.cos_lat) / c);
        lon_rad = (ref.lon_rad + atan2(y_rad * sin_c, c * ref.cos_lat * cos_c - x_rad * ref.sin_lat * sin_c));
    else
        lat_rad = ref.lat_rad;
        lon_rad = ref.lon_rad;
    end

    lat = lat_rad * 180.0 / M_PI;
    lon = lon_rad * 180.0 / M_PI;
    
    out = 0;
end

function [ out, x, y ] = map_projection_project( ref, lat, lon, x, y )
%MAP_PROJECTION_PROJECT
    CONSTANTS_RADIUS_OF_EARTH = 6371000;
    M_DEG_TO_RAD = 0.017453292519943295;
    
    if ( ~map_projection_initialized(ref))
        out = -1;
        return
    end
    
    lat_rad = lat * M_DEG_TO_RAD;
    lon_rad = lon * M_DEG_TO_RAD;

    sin_lat = sin(lat_rad);
    cos_lat = cos(lat_rad);
    cos_d_lon = cos(lon_rad - ref.lon_rad);

    c = acos(ref.sin_lat * sin_lat + ref.cos_lat * cos_lat * cos_d_lon);
    % k = (fabs(c) < DBL_EPSILON) ? 1.0 : (c / sin(c));
    if (abs(c) < eps)
        k = 1.0;
    else
        k = c / sin(c);
    end

    x = k * (ref.cos_lat * sin_lat - ref.sin_lat * cos_lat * cos_d_lon) * CONSTANTS_RADIUS_OF_EARTH;
    y = k * cos_lat * sin(lon_rad - ref.lon_rad) * CONSTANTS_RADIUS_OF_EARTH;

    out = 0;
end

function init = map_projection_initialized( ref )
% MAP_PROJECTION_INITIALIZED
    init = ref.init_done;
end

function [out, ref] = map_projection_init_timestamped(ref, lat_0, lon_0, timestamp) % lat_0, lon_0 are expected to be in correct format: -> 47.1234567 and not 471234567
    M_DEG_TO_RAD = 0.017453292519943295;
	ref.lat_rad = lat_0 * M_DEG_TO_RAD;
	ref.lon_rad = lon_0 * M_DEG_TO_RAD;
	ref.sin_lat = sin(ref.lat_rad);
	ref.cos_lat = cos(ref.lat_rad);

	ref.timestamp = timestamp;
	ref.init_done = double(1);

	out = 0;
end

function [out, lp_block] = block_lowpass_update( input, lp_block )
%BLOCK_LOWPASS_UPADE Update low pass filter
    M_PI = 3.14159265358979323846;
    if (~min(isfinite(lp_block.state)))
		lp_block.state = input;
    end

    b = 2 * M_PI * lp_block.fcut * lp_block.dt;
    a = b / (1 + b);
    lp_block.state = a * input + (1 - a) * lp_block.state;
    out = lp_block.state;
end

function self = initialize_blocks(dt, self)
%INITIALIZE_BLOCKS Initialise low pass blocks
    self.xLowPass.dt = dt;
    self.aglLowPass.dt = dt;
end

function self = setDt( dt, self )
%SETDT Set dt for subblocks
    self.xLowPass.dt = dt;
    self.aglLowPass.dt = dt;
end

%% BlockDelay
% matrix::Matrix<Type, M, N>
function [output, blockDelay] = updateBlockDelay( blockDelay, u )
    LEN = 10;
    % store current value
    blockDelay.h(:,blockDelay.index) = u;

    % delay starts at zero, then increases to LEN
    blockDelay.delay = blockDelay.delay + 1;

    if ( blockDelay.delay > LEN )
        blockDelay.delay = LEN;
    end

    % compute position of delayed value
    j = blockDelay.index - blockDelay.delay;

    if (j < 1)
        j = j + LEN;
    end

    % increment storage position
    blockDelay.index = blockDelay.index + 1;

    if ( blockDelay.index > LEN )
        blockDelay.index  = 1;
    end

    % get delayed value
    output = blockDelay.h(:,j);
end

%% MOCAP
% void BlockLocalPositionEstimator::
function self = mocapInit( self )
%MOCAPINIT Initialise mocap
	% measure
	%Vector<float, n_y_mocap>
	n_y_mocap = 3;
	y = zeros(n_y_mocap, 1);

	[self, success, y] = mocapMeasure( self );

	if ( success ~= 1 )
		self.mocapStats.count = 0;
		return;
	end

	% if finished
	REQ_MOCAP_INIT_COUNT = 1;%20;
	if (self.mocapStats.count > REQ_MOCAP_INIT_COUNT)
		% mavlink_and_console_log_info(&mavlink_log_pub, ['[lpe] mocap position init: '
		% 			     '%5.2f, %5.2f, %5.2f m std %5.2f, %5.2f, %5.2f m'],
		% 			     double(self.mocapStats.getMean()(0)),
		% 			     double(self.mocapStats.getMean()(1)),
		% 			     double(self.mocapStats.getMean()(2)),
		% 			     double(self.mocapStats.getStdDev()(0)),
		% 			     double(self.mocapStats.getStdDev()(1)),
		% 			     double(self.mocapStats.getStdDev()(2)));
		self.sensorTimeout = bitand( self.sensorTimeout, bitcmp( self.SENSOR_MOCAP , 'uint8' ));
		self.sensorFault = bitand( self.sensorFault, bitcmp( self.SENSOR_MOCAP , 'uint8' ));

		if (~self.altOriginInitialized)
			self.altOriginInitialized = 1;
			self.altOrigin = 0;
		end
	end
end

% int BlockLocalPositionEstimator:: % Vector<float, n_y_mocap> &y
function [self, output, y] = mocapMeasure( self )
%MOCAPMEASURE Retrieve mocap measurement
	Y_mocap_x = 1; Y_mocap_y = 2; Y_mocap_z = 3; n_y_mocap = 3;
	y = zeros(n_y_mocap, 1);
	y(Y_mocap_x) = self.sub_mocap.x;
	y(Y_mocap_y) = self.sub_mocap.y;
	y(Y_mocap_z) = self.sub_mocap.z;
	% self.mocapStats.update( y );
	self.mocapStats.count = self.mocapStats.count + 1;
	self.time_last_mocap = self.sub_mocap.timestamp;
	output = 1;
end

% void BlockLocalPositionEstimator::
function self = mocapCorrect( self )
%MOCAPCORRECT Perform correction step with mocap data
	X_x = 1; X_y = 2; X_z = 3; X_vx = 4; X_vy = 5; X_vz = 6;
	X_bx = 7; X_by = 8; X_bz = 9; X_tz = 10; n_x = 10;
	Y_mocap_x = 1; Y_mocap_y = 2; Y_mocap_z = 3; n_y_mocap = 3;

	% measure
	% Vector<float, n_y_mocap> y;
	y = zeros(n_y_mocap, 1);

	[self, success, y] = mocapMeasure( self );

	if ( success ~= 1)
		return;
	end

	% mocap measurement matrix, measures position
	% Matrix<float, n_y_mocap, n_x> C;
	% C.setZero();
	C = zeros( n_y_mocap, n_x );
	C(Y_mocap_x, X_x) = 1;
	C(Y_mocap_y, X_y) = 1;
	C(Y_mocap_z, X_z) = 1;

	% noise matrix
	% Matrix<float, n_y_mocap, n_y_mocap> R;
	% R.setZero();

	R = zeros( n_y_mocap, n_y_mocap );

	% float
	mocap_p_var = self.mocap_p_stddev * self.mocap_p_stddev;
	R(Y_mocap_x, Y_mocap_x) = mocap_p_var;
	R(Y_mocap_y, Y_mocap_y) = mocap_p_var;
	R(Y_mocap_z, Y_mocap_z) = mocap_p_var;

	% residual
	% Matrix<float, n_y_mocap, n_y_mocap> inv<float, n_y_mocap>
	S_I = inv((C * self.P * C') + R);
	% Matrix<float, n_y_mocap, 1>
	r = y - C * self.x;

	% fault detection
	% float
	betaTmp = ( r' * (S_I * r));
	beta1 = betaTmp(1, 1);

	if ( beta1 > self.BETA_TABLE(n_y_mocap) ) 
		if ( ~bitand( self.sensorFault, self.SENSOR_MOCAP ) )
			%mavlink_and_console_log_info(&mavlink_log_pub, "[lpe] mocap fault, beta1 %5.2f", double(beta1));
			self.sensorFault = bitor( self.sensorFault, self.SENSOR_MOCAP );
		end
    elseif bitand(self.sensorFault, self.SENSOR_MOCAP)
		self.sensorFault = bitand( self.sensorFault, bitcmp( self.SENSOR_MOCAP , 'uint8' ));
		%mavlink_and_console_log_info(&mavlink_log_pub, "[lpe] mocap OK");
	end

	% kalman filter correction always
	% Matrix<float, n_x, n_y_mocap>
	K = self.P * C' * S_I;
	% Vector<float, n_x>
	dx = K * r;
	self.x = self.x + dx;
	self.P = self.P - K * C * self.P;
end

% void BlockLocalPositionEstimator::
function self = mocapCheckTimeout( self )
%MOCAPCHECKTIMEOUT Check if mocap has timed out
	MOCAP_TIMEOUT = 200000; % 0.2 s

	if ((self.timeStamp - self.time_last_mocap) > MOCAP_TIMEOUT)
		if (~bitand(self.sensorTimeout, self.SENSOR_MOCAP))
			self.sensorTimeout = bitor( self.sensorTimeout, self.SENSOR_MOCAP ); % |=
			% self.mocapStats.reset();
			self.mocapStats.count = 0;
			% mavlink_and_console_log_info(mavlink_log_pub, '[lpe] mocap timeout ');
		end
	end
end

%% BARO
% void BlockLocalPositionEstimator::
function self = baroInit( self )
%BAROINIT Initialise barometer
	% measure
	y = 0;

	[self, success, y] = baroMeasure( self );

	if ( success ~= 1 )
		self.baroStats.count = 0;
		self.baroStats.total = 0;
		return;
	end

	% if finished
	REQ_BARO_INIT_COUNT = 100;
	if ( self.baroStats.count > REQ_BARO_INIT_COUNT )
		self.baroAltOrigin = self.baroStats.total / self.baroStats.count; % TAKE CARE OF THIS
		% mavlink_and_console_log_info(&mavlink_log_pub,
		% 			     '[lpe] baro init %d m std %d cm',
		% 			     (int)self.baroStats.getMean()(0),
		% 			     (int)(100 * self.baroStats.getStdDev()(0)));
		self.sensorTimeout = bitand( self.sensorTimeout, bitcmp( self.SENSOR_BARO , 'uint8' ));
		self.sensorFault = bitand( self.sensorFault, bitcmp( self.SENSOR_BARO , 'uint8' ));

		if (~self.altOriginInitialized)
			self.altOriginInitialized = 1;
			self.altOrigin = self.baroAltOrigin;
		end
	end
end

% int BlockLocalPositionEstimator:: Vector<float, n_y_baro> &y
function [self, output, y ] = baroMeasure( self )
%BAROMEASURE Retrieve barometer measurement
	%measure
	y = 0;
	y = self.sub_sensor.baro_alt_meter;
	self.baroStats.count = self.baroStats.count + 1; %update(y);
	self.baroStats.total = self.baroStats.total + y;
	self.time_last_baro = self.timeStamp;
	output = 1;
end

% void BlockLocalPositionEstimator::
function self = baroCorrect( self )
%BAROCORRECT Correction step for barometer measurement
	X_x = 1; X_y = 2; X_z = 3; X_vx = 4; X_vy = 5; X_vz = 6;
	X_bx = 7; X_by = 8; X_bz = 9; X_tz = 10; n_x = 10;
	Y_baro_z = 1; n_y_baro = 1;

	% measure
	%Vector<float, n_y_baro>
	y = 0;

	[self, success, y] = baroMeasure( self );

	if ( success ~= 1 )
		self.baroStats.count = 0;
		self.baroStats.total = 0;
		return;
	end

	% subtract baro origin alt
	y = y - self.baroAltOrigin;

	% baro measurement matrix
	% Matrix<float, n_y_baro, n_x> C;
	% C.setZero();
	C = zeros( n_y_baro, n_x );

	C(Y_baro_z, X_z) = -1; % measured altitude, negative down dir.

	% Matrix<float, n_y_baro, n_y_baro> R;
	% R.setZero();
	R = zeros( n_y_baro, n_y_baro );
	R(1, 1) = self.baro_stddev * self.baro_stddev;

	% residual
	% Matrix<float, n_y_baro, n_y_baro> <float, n_y_baro>
	S_I = inv((C * self.P * C') + R);
	% Vector<float, n_y_baro>
	r = y - (C * self.x);

	% fault detection
